simulink model "Noordergraaf_Rideout_2021b"  (R2021b)
settings: Solver=FixedStepAuto  StartTime=0.0  StopTime=stop_time  FixedStep=sample_time  RelTol=1e-3
undefined symbols (not defined in the file or in its folder): C, L, R, R_105, R_26, R_29, R_34, R_35, R_60, R_61, R_64, R_65, R_66, R_70, R_82, R_84, R_88, R_90, R_AT, R_SA, sample_time
libraries: ee_lib x421, fl_lib x87, nesl_utility x57, simulink x1
(part 1 of 9)
settings Model: Creator=jorge  LastModifiedBy=jorge
settings SolverCC: InitialStep=sample_time

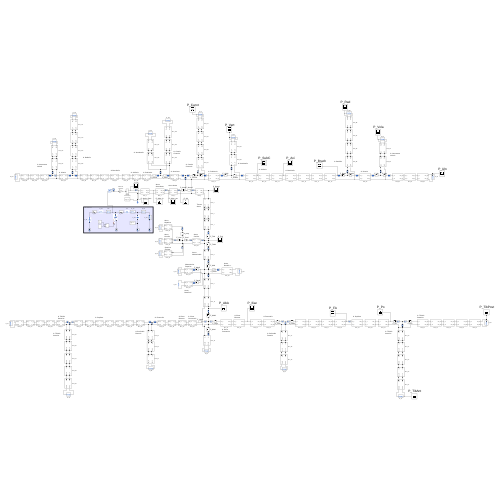
[thumbnail: Simulink's stored preview of the top-level diagram]
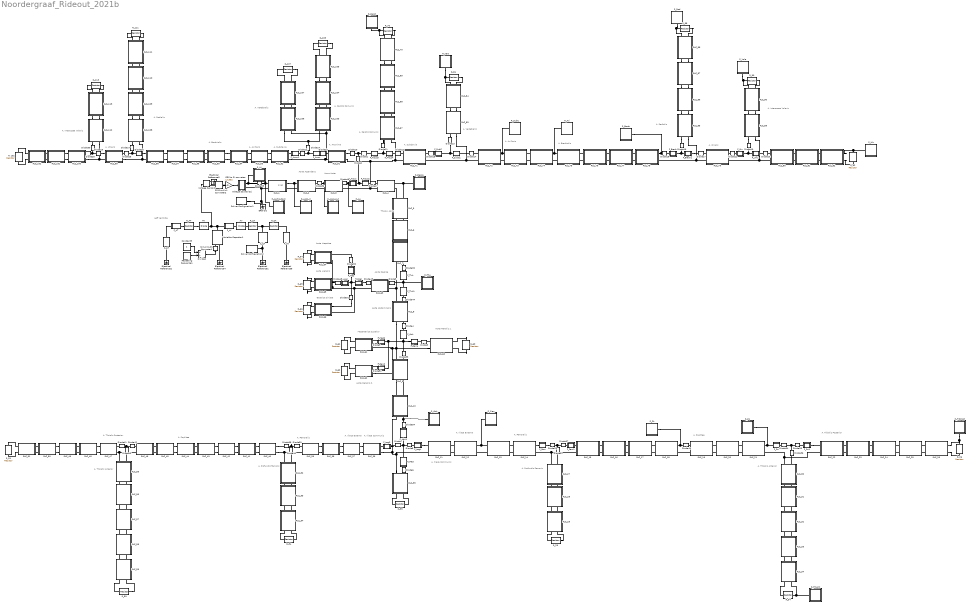
== system Noordergraaf_Rideout_2021b ==
  note: Aorta
      | Ascendens
  note: ones
  note: Arcus Aorta
  note: Thorax
      | Aorta
  note: Aorta
      | Coelica
  note: Gastrica
      | Sinistra
  note: Aorta
      | Lienalis
  note: Aorta
      | Hepatica
  note: Aorta
      | Abdominalis
  note: Aorta
      | Renalis d.
  note: Mesenterica
      | Superior
  note: Aorta
      | Renalis s.
  note: A. Iliaca
      | Communis
  note: A. Iliaca
      | Externa
  note: A. Femoralis
  note: A. Profundis
      | Femoris
  note: A. Tibialis
      | Anterior
  note: A. Poplitea
  note: A. Tibialis
      | Posterior
  note: A. Iliaca
      | Communis
  note: A. Iliaca
      | Externa
  note: A. Femoralis
  note: A. Poplitea
  note: A. Tibialis
      | Posterior
  note: A. Profundis
      | Femoris
  note: A. Tibialis
      | Anterior
  note: A. Carotis
      | Comunis
  note: A. Ulnaris
  note: A. Brachialis
  note: A. Subclavia
  note: A. Axillaris
  note: A. Radialis
  note: A. Subclavia
  note: A. Axillaris
  note: A. Brachialis
  note: A. Ulnaris
  note: A. Vertebralis
  note: A. Carotis
      | Comunis
  note: A. Vertebralis
  note: A. Interossea
      | Volaris
  note: A. Interossea
      | Volaris
  note: A. Radialis
  note: A. Anonima
  note: Left Ventricle
  " P_AA" : Subsystem
      settings: PortSchema="{\"entries\":[{\"content\":{\"sides\":[{\"content\":{\"connectorIds\":[]},\"type\":\"ConnectorPlacement.EquallySpacedRectSide\",\"uuid\":\"a76c572b-3baf-4a16-ab2f-87d419d93200\"},{\"content\":{\"connectorIds\":[],\"side\":\"RIGHT\"},\"type\":\"ConnectorPlacement.EquallySpacedRectSide\",\"uuid\":\"88de64cb-36a9-4b54-8774-bd24fb5aa84a\"},{\"content\":{\"connectorIds\":[\"LConn1\"],\"side\":\"TOP\"},\"type\":\"ConnectorPlacement.EquallySpacedRectSide\",\"uuid\":\"3a1c039d-3fc9-4c0f-9a54-0653a75cef5f\"},{\"content\":{\"connectorIds\":[],\"side\":\"HIDDEN\"},\"type\":\"ConnectorPlacement.EquallySpacedRectSide\",\"uuid\":\"5afc8217-ede4-4d55-8a13-208761f7f032\"}]},\"type\":\"ConnectorPlacement.EquallySpacedConnector\",\"uuid\":\"92a25d9f-67d7-41a2-ac65-068fc761adb7\"}],\"packageUris\":[\"http://schema.mathworks.com/mf0/Connector/R2020b\"],\"version\":\"1.0\"}"
      mask Display: image('$imagefile');
  " P_AAsc_in" : Subsystem
      settings: PortSchema="{\"entries\":[{\"content\":{\"sides\":[{\"content\":{\"connectorIds\":[]},\"type\":\"ConnectorPlacement.EquallySpacedRectSide\",\"uuid\":\"a76c572b-3baf-4a16-ab2f-87d419d93200\"},{\"content\":{\"connectorIds\":[],\"side\":\"RIGHT\"},\"type\":\"ConnectorPlacement.EquallySpacedRectSide\",\"uuid\":\"88de64cb-36a9-4b54-8774-bd24fb5aa84a\"},{\"content\":{\"connectorIds\":[\"LConn1\"],\"side\":\"TOP\"},\"type\":\"ConnectorPlacement.EquallySpacedRectSide\",\"uuid\":\"3a1c039d-3fc9-4c0f-9a54-0653a75cef5f\"},{\"content\":{\"connectorIds\":[],\"side\":\"HIDDEN\"},\"type\":\"ConnectorPlacement.EquallySpacedRectSide\",\"uuid\":\"5afc8217-ede4-4d55-8a13-208761f7f032\"}]},\"type\":\"ConnectorPlacement.EquallySpacedConnector\",\"uuid\":\"92a25d9f-67d7-41a2-ac65-068fc761adb7\"}],\"packageUris\":[\"http://schema.mathworks.com/mf0/Connector/R2020b\"],\"version\":\"1.0\"}"
      mask Display: image('$imagefile'); % Use "Edit Image" on toolstrip to change.
  " P_AAsc_out" : Subsystem
      settings: PortSchema="{\"entries\":[{\"content\":{\"sides\":[{\"content\":{\"connectorIds\":[]},\"type\":\"ConnectorPlacement.EquallySpacedRectSide\",\"uuid\":\"a76c572b-3baf-4a16-ab2f-87d419d93200\"},{\"content\":{\"connectorIds\":[],\"side\":\"RIGHT\"},\"type\":\"ConnectorPlacement.EquallySpacedRectSide\",\"uuid\":\"88de64cb-36a9-4b54-8774-bd24fb5aa84a\"},{\"content\":{\"connectorIds\":[\"LConn1\"],\"side\":\"TOP\"},\"type\":\"ConnectorPlacement.EquallySpacedRectSide\",\"uuid\":\"3a1c039d-3fc9-4c0f-9a54-0653a75cef5f\"},{\"content\":{\"connectorIds\":[],\"side\":\"HIDDEN\"},\"type\":\"ConnectorPlacement.EquallySpacedRectSide\",\"uuid\":\"5afc8217-ede4-4d55-8a13-208761f7f032\"}]},\"type\":\"ConnectorPlacement.EquallySpacedConnector\",\"uuid\":\"92a25d9f-67d7-41a2-ac65-068fc761adb7\"}],\"packageUris\":[\"http://schema.mathworks.com/mf0/Connector/R2020b\"],\"version\":\"1.0\"}"
      mask Display: image('$imagefile'); % Use "Edit Image" on toolstrip to change.
  " P_AbA" : Subsystem
      settings: PortSchema="{\"entries\":[{\"content\":{\"sides\":[{\"content\":{\"connectorIds\":[]},\"type\":\"ConnectorPlacement.EquallySpacedRectSide\",\"uuid\":\"a76c572b-3baf-4a16-ab2f-87d419d93200\"},{\"content\":{\"connectorIds\":[],\"side\":\"RIGHT\"},\"type\":\"ConnectorPlacement.EquallySpacedRectSide\",\"uuid\":\"88de64cb-36a9-4b54-8774-bd24fb5aa84a\"},{\"content\":{\"connectorIds\":[\"LConn1\"],\"side\":\"TOP\"},\"type\":\"ConnectorPlacement.EquallySpacedRectSide\",\"uuid\":\"3a1c039d-3fc9-4c0f-9a54-0653a75cef5f\"},{\"content\":{\"connectorIds\":[],\"side\":\"HIDDEN\"},\"type\":\"ConnectorPlacement.EquallySpacedRectSide\",\"uuid\":\"5afc8217-ede4-4d55-8a13-208761f7f032\"}]},\"type\":\"ConnectorPlacement.EquallySpacedConnector\",\"uuid\":\"92a25d9f-67d7-41a2-ac65-068fc761adb7\"}],\"packageUris\":[\"http://schema.mathworks.com/mf0/Connector/R2020b\"],\"version\":\"1.0\"}"
      mask Display: image('$imagefile'); % Use "Edit Image" on toolstrip to change.
  " P_Aortic_Root" : Subsystem
      settings: PortSchema="{\"entries\":[{\"content\":{\"sides\":[{\"content\":{\"connectorIds\":[]},\"type\":\"ConnectorPlacement.EquallySpacedRectSide\",\"uuid\":\"a76c572b-3baf-4a16-ab2f-87d419d93200\"},{\"content\":{\"connectorIds\":[],\"side\":\"RIGHT\"},\"type\":\"ConnectorPlacement.EquallySpacedRectSide\",\"uuid\":\"88de64cb-36a9-4b54-8774-bd24fb5aa84a\"},{\"content\":{\"connectorIds\":[\"LConn1\"],\"side\":\"TOP\"},\"type\":\"ConnectorPlacement.EquallySpacedRectSide\",\"uuid\":\"3a1c039d-3fc9-4c0f-9a54-0653a75cef5f\"},{\"content\":{\"connectorIds\":[],\"side\":\"HIDDEN\"},\"type\":\"ConnectorPlacement.EquallySpacedRectSide\",\"uuid\":\"5afc8217-ede4-4d55-8a13-208761f7f032\"}]},\"type\":\"ConnectorPlacement.EquallySpacedConnector\",\"uuid\":\"92a25d9f-67d7-41a2-ac65-068fc761adb7\"}],\"packageUris\":[\"http://schema.mathworks.com/mf0/Connector/R2020b\"],\"version\":\"1.0\"}"
      mask Display: image('$imagefile'); % Use "Edit Image" on toolstrip to change.
  " P_Axi" : Subsystem
      settings: PortSchema="{\"entries\":[{\"content\":{\"sides\":[{\"content\":{\"connectorIds\":[]},\"type\":\"ConnectorPlacement.EquallySpacedRectSide\",\"uuid\":\"a76c572b-3baf-4a16-ab2f-87d419d93200\"},{\"content\":{\"connectorIds\":[],\"side\":\"RIGHT\"},\"type\":\"ConnectorPlacement.EquallySpacedRectSide\",\"uuid\":\"88de64cb-36a9-4b54-8774-bd24fb5aa84a\"},{\"content\":{\"connectorIds\":[\"LConn1\"],\"side\":\"TOP\"},\"type\":\"ConnectorPlacement.EquallySpacedRectSide\",\"uuid\":\"3a1c039d-3fc9-4c0f-9a54-0653a75cef5f\"},{\"content\":{\"connectorIds\":[],\"side\":\"BOTTOM\"},\"type\":\"ConnectorPlacement.EquallySpacedRectSide\",\"uuid\":\"16f5eb9b-ee63-4f34-9118-7825bbfe571f\"},{\"content\":{\"connectorIds\":[],\"side\":\"HIDDEN\"},\"type\":\"ConnectorPlacement.EquallySpacedRectSide\",\"uuid\":\"5afc8217-ede4-4d55-8a13-208761f7f032\"}]},\"type\":\"ConnectorPlacement.EquallySpacedConnector\",\"uuid\":\"92a25d9f-67d7-41a2-ac65-068fc761adb7\"}],\"packageUris\":[\"http://schema.mathworks.com/mf0/Connector/R2020b\"],\"version\":\"1.0\"}"
      mask Display: image('$imagefile'); % Use "Edit Image" on toolstrip to change.
  " P_Brach" : Subsystem
      settings: PortSchema="{\"entries\":[{\"content\":{\"sides\":[{\"content\":{\"connectorIds\":[]},\"type\":\"ConnectorPlacement.EquallySpacedRectSide\",\"uuid\":\"a76c572b-3baf-4a16-ab2f-87d419d93200\"},{\"content\":{\"connectorIds\":[],\"side\":\"RIGHT\"},\"type\":\"ConnectorPlacement.EquallySpacedRectSide\",\"uuid\":\"88de64cb-36a9-4b54-8774-bd24fb5aa84a\"},{\"content\":{\"connectorIds\":[],\"side\":\"TOP\"},\"type\":\"ConnectorPlacement.EquallySpacedRectSide\",\"uuid\":\"3a1c039d-3fc9-4c0f-9a54-0653a75cef5f\"},{\"content\":{\"connectorIds\":[\"RConn1\"],\"side\":\"BOTTOM\"},\"type\":\"ConnectorPlacement.EquallySpacedRectSide\",\"uuid\":\"16f5eb9b-ee63-4f34-9118-7825bbfe571f\"},{\"content\":{\"connectorIds\":[],\"side\":\"HIDDEN\"},\"type\":\"ConnectorPlacement.EquallySpacedRectSide\",\"uuid\":\"5afc8217-ede4-4d55-8a13-208761f7f032\"}]},\"type\":\"ConnectorPlacement.EquallySpacedConnector\",\"uuid\":\"92a25d9f-67d7-41a2-ac65-068fc761adb7\"}],\"packageUris\":[\"http://schema.mathworks.com/mf0/Connector/R2020b\"],\"version\":\"1.0\"}"
      mask Display: image('$imagefile'); % Use "Edit Image" on toolstrip to change.
  " P_Carot" : Subsystem
      mask Display: image('$imagefile'); % Use "Edit Image" on toolstrip to change.
  " P_DescA" : Subsystem
      settings: PortSchema="{\"entries\":[{\"content\":{\"sides\":[{\"content\":{\"connectorIds\":[]},\"type\":\"ConnectorPlacement.EquallySpacedRectSide\",\"uuid\":\"a76c572b-3baf-4a16-ab2f-87d419d93200\"},{\"content\":{\"connectorIds\":[],\"side\":\"RIGHT\"},\"type\":\"ConnectorPlacement.EquallySpacedRectSide\",\"uuid\":\"88de64cb-36a9-4b54-8774-bd24fb5aa84a\"},{\"content\":{\"connectorIds\":[\"LConn1\"],\"side\":\"TOP\"},\"type\":\"ConnectorPlacement.EquallySpacedRectSide\",\"uuid\":\"3a1c039d-3fc9-4c0f-9a54-0653a75cef5f\"},{\"content\":{\"connectorIds\":[],\"side\":\"HIDDEN\"},\"type\":\"ConnectorPlacement.EquallySpacedRectSide\",\"uuid\":\"5afc8217-ede4-4d55-8a13-208761f7f032\"}]},\"type\":\"ConnectorPlacement.EquallySpacedConnector\",\"uuid\":\"92a25d9f-67d7-41a2-ac65-068fc761adb7\"}],\"packageUris\":[\"http://schema.mathworks.com/mf0/Connector/R2020b\"],\"version\":\"1.0\"}"
      mask Display: image('$imagefile'); % Use "Edit Image" on toolstrip to change.
  " P_FA" : Subsystem
      settings: PortSchema="{\"entries\":[{\"content\":{\"sides\":[{\"content\":{\"connectorIds\":[]},\"type\":\"ConnectorPlacement.EquallySpacedRectSide\",\"uuid\":\"a76c572b-3baf-4a16-ab2f-87d419d93200\"},{\"content\":{\"connectorIds\":[],\"side\":\"RIGHT\"},\"type\":\"ConnectorPlacement.EquallySpacedRectSide\",\"uuid\":\"88de64cb-36a9-4b54-8774-bd24fb5aa84a\"},{\"content\":{\"connectorIds\":[],\"side\":\"TOP\"},\"type\":\"ConnectorPlacement.EquallySpacedRectSide\",\"uuid\":\"3a1c039d-3fc9-4c0f-9a54-0653a75cef5f\"},{\"content\":{\"connectorIds\":[\"RConn1\"],\"side\":\"BOTTOM\"},\"type\":\"ConnectorPlacement.EquallySpacedRectSide\",\"uuid\":\"041fbf42-3c46-4830-b301-418dfd34a912\"},{\"content\":{\"connectorIds\":[],\"side\":\"HIDDEN\"},\"type\":\"ConnectorPlacement.EquallySpacedRectSide\",\"uuid\":\"5afc8217-ede4-4d55-8a13-208761f7f032\"}]},\"type\":\"ConnectorPlacement.EquallySpacedConnector\",\"uuid\":\"92a25d9f-67d7-41a2-ac65-068fc761adb7\"}],\"packageUris\":[\"http://schema.mathworks.com/mf0/Connector/R2020b\"],\"version\":\"1.0\"}"
      mask Display: image('$imagefile'); % Use "Edit Image" on toolstrip to change.
  " P_Iliac" : Subsystem
      settings: PortSchema="{\"entries\":[{\"content\":{\"sides\":[{\"content\":{\"connectorIds\":[]},\"type\":\"ConnectorPlacement.EquallySpacedRectSide\",\"uuid\":\"a76c572b-3baf-4a16-ab2f-87d419d93200\"},{\"content\":{\"connectorIds\":[],\"side\":\"RIGHT\"},\"type\":\"ConnectorPlacement.EquallySpacedRectSide\",\"uuid\":\"88de64cb-36a9-4b54-8774-bd24fb5aa84a\"},{\"content\":{\"connectorIds\":[\"LConn1\"],\"side\":\"TOP\"},\"type\":\"ConnectorPlacement.EquallySpacedRectSide\",\"uuid\":\"3a1c039d-3fc9-4c0f-9a54-0653a75cef5f\"},{\"content\":{\"connectorIds\":[],\"side\":\"BOTTOM\"},\"type\":\"ConnectorPlacement.EquallySpacedRectSide\",\"uuid\":\"041fbf42-3c46-4830-b301-418dfd34a912\"},{\"content\":{\"connectorIds\":[],\"side\":\"HIDDEN\"},\"type\":\"ConnectorPlacement.EquallySpacedRectSide\",\"uuid\":\"5afc8217-ede4-4d55-8a13-208761f7f032\"}]},\"type\":\"ConnectorPlacement.EquallySpacedConnector\",\"uuid\":\"92a25d9f-67d7-41a2-ac65-068fc761adb7\"}],\"packageUris\":[\"http://schema.mathworks.com/mf0/Connector/R2020b\"],\"version\":\"1.0\"}"
      mask Display: image('$imagefile'); % Use "Edit Image" on toolstrip to change.
  " P_LV" : Subsystem
      settings: PortSchema="{\"entries\":[{\"content\":{\"sides\":[{\"content\":{\"connectorIds\":[]},\"type\":\"ConnectorPlacement.EquallySpacedRectSide\",\"uuid\":\"a76c572b-3baf-4a16-ab2f-87d419d93200\"},{\"content\":{\"connectorIds\":[],\"side\":\"RIGHT\"},\"type\":\"ConnectorPlacement.EquallySpacedRectSide\",\"uuid\":\"88de64cb-36a9-4b54-8774-bd24fb5aa84a\"},{\"content\":{\"connectorIds\":[\"LConn1\"],\"side\":\"TOP\"},\"type\":\"ConnectorPlacement.EquallySpacedRectSide\",\"uuid\":\"3a1c039d-3fc9-4c0f-9a54-0653a75cef5f\"},{\"content\":{\"connectorIds\":[],\"side\":\"HIDDEN\"},\"type\":\"ConnectorPlacement.EquallySpacedRectSide\",\"uuid\":\"5afc8217-ede4-4d55-8a13-208761f7f032\"}]},\"type\":\"ConnectorPlacement.EquallySpacedConnector\",\"uuid\":\"92a25d9f-67d7-41a2-ac65-068fc761adb7\"}],\"packageUris\":[\"http://schema.mathworks.com/mf0/Connector/R2020b\"],\"version\":\"1.0\"}"
      mask Display: image('$imagefile'); % Use "Edit Image" on toolstrip to change.
  " P_Po" : Subsystem
      settings: PortSchema="{\"entries\":[{\"content\":{\"sides\":[{\"content\":{\"connectorIds\":[]},\"type\":\"ConnectorPlacement.EquallySpacedRectSide\",\"uuid\":\"a76c572b-3baf-4a16-ab2f-87d419d93200\"},{\"content\":{\"connectorIds\":[],\"side\":\"RIGHT\"},\"type\":\"ConnectorPlacement.EquallySpacedRectSide\",\"uuid\":\"88de64cb-36a9-4b54-8774-bd24fb5aa84a\"},{\"content\":{\"connectorIds\":[],\"side\":\"TOP\"},\"type\":\"ConnectorPlacement.EquallySpacedRectSide\",\"uuid\":\"3a1c039d-3fc9-4c0f-9a54-0653a75cef5f\"},{\"content\":{\"connectorIds\":[\"RConn1\"],\"side\":\"BOTTOM\"},\"type\":\"ConnectorPlacement.EquallySpacedRectSide\",\"uuid\":\"041fbf42-3c46-4830-b301-418dfd34a912\"},{\"content\":{\"connectorIds\":[],\"side\":\"HIDDEN\"},\"type\":\"ConnectorPlacement.EquallySpacedRectSide\",\"uuid\":\"5afc8217-ede4-4d55-8a13-208761f7f032\"}]},\"type\":\"ConnectorPlacement.EquallySpacedConnector\",\"uuid\":\"92a25d9f-67d7-41a2-ac65-068fc761adb7\"}],\"packageUris\":[\"http://schema.mathworks.com/mf0/Connector/R2020b\"],\"version\":\"1.0\"}"
      mask Display: image('$imagefile'); % Use "Edit Image" on toolstrip to change.
  " P_Rad" : Subsystem
      mask Display: image('$imagefile'); % Use "Edit Image" on toolstrip to change.
  " P_SubC" : Subsystem
      settings: PortSchema="{\"entries\":[{\"content\":{\"sides\":[{\"content\":{\"connectorIds\":[]},\"type\":\"ConnectorPlacement.EquallySpacedRectSide\",\"uuid\":\"a76c572b-3baf-4a16-ab2f-87d419d93200\"},{\"content\":{\"connectorIds\":[],\"side\":\"RIGHT\"},\"type\":\"ConnectorPlacement.EquallySpacedRectSide\",\"uuid\":\"88de64cb-36a9-4b54-8774-bd24fb5aa84a\"},{\"content\":{\"connectorIds\":[\"LConn1\"],\"side\":\"TOP\"},\"type\":\"ConnectorPlacement.EquallySpacedRectSide\",\"uuid\":\"3a1c039d-3fc9-4c0f-9a54-0653a75cef5f\"},{\"content\":{\"connectorIds\":[],\"side\":\"BOTTOM\"},\"type\":\"ConnectorPlacement.EquallySpacedRectSide\",\"uuid\":\"16f5eb9b-ee63-4f34-9118-7825bbfe571f\"},{\"content\":{\"connectorIds\":[],\"side\":\"HIDDEN\"},\"type\":\"ConnectorPlacement.EquallySpacedRectSide\",\"uuid\":\"5afc8217-ede4-4d55-8a13-208761f7f032\"}]},\"type\":\"ConnectorPlacement.EquallySpacedConnector\",\"uuid\":\"92a25d9f-67d7-41a2-ac65-068fc761adb7\"}],\"packageUris\":[\"http://schema.mathworks.com/mf0/Connector/R2020b\"],\"version\":\"1.0\"}"
      mask Display: image('$imagefile'); % Use "Edit Image" on toolstrip to change.
  " P_ThA" : Subsystem
      settings: PortSchema="{\"entries\":[{\"content\":{\"sides\":[{\"content\":{\"connectorIds\":[]},\"type\":\"ConnectorPlacement.EquallySpacedRectSide\",\"uuid\":\"a76c572b-3baf-4a16-ab2f-87d419d93200\"},{\"content\":{\"connectorIds\":[],\"side\":\"RIGHT\"},\"type\":\"ConnectorPlacement.EquallySpacedRectSide\",\"uuid\":\"88de64cb-36a9-4b54-8774-bd24fb5aa84a\"},{\"content\":{\"connectorIds\":[\"LConn1\"],\"side\":\"TOP\"},\"type\":\"ConnectorPlacement.EquallySpacedRectSide\",\"uuid\":\"3a1c039d-3fc9-4c0f-9a54-0653a75cef5f\"},{\"content\":{\"connectorIds\":[],\"side\":\"HIDDEN\"},\"type\":\"ConnectorPlacement.EquallySpacedRectSide\",\"uuid\":\"5afc8217-ede4-4d55-8a13-208761f7f032\"}]},\"type\":\"ConnectorPlacement.EquallySpacedConnector\",\"uuid\":\"92a25d9f-67d7-41a2-ac65-068fc761adb7\"}],\"packageUris\":[\"http://schema.mathworks.com/mf0/Connector/R2020b\"],\"version\":\"1.0\"}"
      mask Display: image('$imagefile'); % Use "Edit Image" on toolstrip to change.
  " P_TibAnt" : Subsystem
      settings: PortSchema="{\"entries\":[{\"content\":{\"sides\":[{\"content\":{\"connectorIds\":[]},\"type\":\"ConnectorPlacement.EquallySpacedRectSide\",\"uuid\":\"efa007d6-45f4-4edc-b08d-571edfadacea\"},{\"content\":{\"connectorIds\":[],\"side\":\"RIGHT\"},\"type\":\"ConnectorPlacement.EquallySpacedRectSide\",\"uuid\":\"9590d5ff-e9bb-4f62-8234-4beabe73ec5b\"},{\"content\":{\"connectorIds\":[\"LConn1\"],\"side\":\"TOP\"},\"type\":\"ConnectorPlacement.EquallySpacedRectSide\",\"uuid\":\"6b36768b-9c7e-47c9-8a74-9f42572fa7f1\"}]},\"type\":\"ConnectorPlacement.EquallySpacedConnector\",\"uuid\":\"e0d20f9b-b643-4fc3-baf2-1c11480af55a\"}],\"packageUris\":[\"http://schema.mathworks.com/mf0/Connector/R2020b\"],\"version\":\"1.0\"}"
      mask Display: image('$imagefile'); % Use "Edit Image" on toolstrip to change.
  " P_TibPost" : Subsystem
      mask Display: image('$imagefile'); % Use "Edit Image" on toolstrip to change.
  " P_Uln" : Subsystem
      settings: PortSchema="{\"entries\":[{\"content\":{\"sides\":[{\"content\":{\"connectorIds\":[]},\"type\":\"ConnectorPlacement.EquallySpacedRectSide\",\"uuid\":\"a76c572b-3baf-4a16-ab2f-87d419d93200\"},{\"content\":{\"connectorIds\":[],\"side\":\"RIGHT\"},\"type\":\"ConnectorPlacement.EquallySpacedRectSide\",\"uuid\":\"88de64cb-36a9-4b54-8774-bd24fb5aa84a\"},{\"content\":{\"connectorIds\":[\"LConn1\"],\"side\":\"TOP\"},\"type\":\"ConnectorPlacement.EquallySpacedRectSide\",\"uuid\":\"3a1c039d-3fc9-4c0f-9a54-0653a75cef5f\"},{\"content\":{\"connectorIds\":[],\"side\":\"BOTTOM\"},\"type\":\"ConnectorPlacement.EquallySpacedRectSide\",\"uuid\":\"16f5eb9b-ee63-4f34-9118-7825bbfe571f\"},{\"content\":{\"connectorIds\":[],\"side\":\"HIDDEN\"},\"type\":\"ConnectorPlacement.EquallySpacedRectSide\",\"uuid\":\"5afc8217-ede4-4d55-8a13-208761f7f032\"}]},\"type\":\"ConnectorPlacement.EquallySpacedConnector\",\"uuid\":\"92a25d9f-67d7-41a2-ac65-068fc761adb7\"}],\"packageUris\":[\"http://schema.mathworks.com/mf0/Connector/R2020b\"],\"version\":\"1.0\"}"
      mask Display: image('$imagefile'); % Use "Edit Image" on toolstrip to change.
  " P_Vert" : Subsystem
      mask Display: image('$imagefile'); % Use "Edit Image" on toolstrip to change.
  " P_Vola" : Subsystem
      mask Display: image('$imagefile'); % Use "Edit Image" on toolstrip to change.
  AV : fl_lib/Electrical/Electrical Elements/Diode  Vf=1 V  Ron=10^(-3) Ohm  Goff=1e-8 1/Ohm  i_specify=off  i_priority=None  i=0 A  i_nominal_specify=off  i_nominal_unit=A  i_nominal_value=1  v_specify=off  v_priority=None  v=0 V  v_nominal_specify=off  v_nominal_unit=V  v_nominal_value=1
  CGS to SI converter : Gain  Gain=1/1332
  C_CA : fl_lib/Electrical/Electrical Elements/Capacitor  c=C_CA F  r=0 Ohm  g=0 1/Ohm  i_specify=off  i_priority=None  i=0 A  i_nominal_specify=off  i_nominal_unit=A  i_nominal_value=220  v_specify=off  v_priority=None  v=0 V  v_nominal_specify=off  v_nominal_unit=V  v_nominal_value=1  vc_specify=off  vc_priority=High  vc=0 V  vc_nominal_specify=off  vc_nominal_unit=V  vc_nominal_value=1
  Constant5 : Constant  SampleTime=sample_time
  Diode{1..56} (56 alike) : ee_lib/Semiconductors & Converters/Diode  ModelType=ee.enum.diode.modelType.pwl  TableType=ee.enum.diode.tableType.IfMat  IfMat=[.07, .12, .19, 1.75, 4.24, 7.32, 11.2; .16, .3, .72, 2.14, 5.02, 8.35, 13.12] A  VfMat=[.9, 1.15, 1.25, 1.5, 1.75, 2.17, 2.6, 2.85; .58, .68, .75, 1.1, 1.38, 1.77, 2.27, 2.7] V  TjVec=[25, 125] degC  VfVec=[.5, .7, .9, 1.3, 1.7, 2.1, 2.5] V  IfVec=[.1, .2, .5, 1, 2, 4, 7, 10] A  Vf=0.6 V  Ron=0.3 Ohm  Goff=1e-8 S  prmExp=ee.enum.diode.expParam.useTwo  I12=[.0137, .545] A  V12=[.6, .7] V  RS=0 Ohm  Tmeas=25 degC  IS=1e-12 A  ec=1  I1=0.0137 A  V1=0.6 V  N_series=1  N_parallel=1  ZenerEnable=false  Rz=0.3 Ohm  BV=inf V  C_param=ee.enum.diode.capParam.fixed  CJ=5 pF  CJ0=5 pF  Vvec=[.1, 10, 100] V  Cvec=[3.5, 1, .4] pF  VJ=1 V  Mgrad=0.5  FC=0.5  Q_param=ee.enum.diode.recoveryParam.off  iRM=-7.15 A  iF=4 A  didt=-750 A/us  trr_factor=3  trr=115 ns  Qrr=150 nA*s  Vr=-600 V  Ls=150 nH  Erec=0.03 J  TT=50 ns  tau=100 ns  T_param=ee.enum.diode.temperatureParam.off  Tdevice=25 degC  I1_T2=0.245 A  V1_T2=0.5 V  IS_T2=1.25e-7 A  Tmeas2=125 degC  XTI_param=ee.enum.diode.xtiParam.pn  XTI=3  EG_param=ee.enum.diode.egapParam.material_si  EG=1.11 eV  dBVdT=0 V/K  enable_faults=ee.enum.enable.no  fault_action=simscape.enum.assert.action.none  fault_types=ee.enum.diode.faults.open  tau_fault=1e-3 s  IfMat_faulted=[.07, .12, .19, 1.75, 4.24, 7.32, 11.2; .16, .3, .72, 2.14, 4.02, 6.35, 9.12] A  VfMat_faulted=[.9, 1.15, 1.25, 1.5, 1.75, 2.17, 2.6, 2.85; .58, .68, .75, 1.1, 1.38, 1.77, 2.27, 2.7] V  VfVec_faulted=[.5, .7, .9, 1.3, 1.7, 2.1, 2.5] V  IfVec_faulted=[.1, .2, .5, 1, 2, 4, 7, 10] A  Ropen_faulted=1000 Ohm  Gshort_faulted=1000 1/Ohm  Vf_faulted=0.6 V  Ron_faulted=0.3 Ohm  Goff_faulted=1e-8 S  I12_faulted=[.0137, .545] A  V12_faulted=[.6, .7] V  IS_faulted=1e-12 A  ec_faulted=1  I1_faulted=0.0137 A  V1_faulted=0.6 V  RS_faulted=0 Ohm  Rz_faulted=0.3 Ohm  BV_faulted=inf V  Cscale_faulted=100  fault_trigger=ee.enum.faults.faultTrigger.temporal  t_fault=inf s  max_permissible_voltage=inf V  n_fail_on_voltage=1  max_permissible_current=inf A  t_fail_on_current=1 s  max_permissible_dVdt=inf V/s  enable_fault_input=simscape.enum.onoff.off  i_specify=off  i_priority=None  i=0 A  i_nominal_specify=off  i_nominal_unit=A  i_nominal_value=1  v_specify=off  v_priority=None  v=0 V  v_nominal_specify=off  v_nominal_unit=V  v_nominal_value=1  v_capacitor_specify=off  v_capacitor_priority=None  v_capacitor=0 V  v_capacitor_nominal_specify=off  v_capacitor_nominal_unit=V  v_capacitor_nominal_value=1  faulted_specify=off  faulted_priority=None  faulted=0  faulted_nominal_specify=off  faulted_nominal_unit=1  faulted_nominal_value=1  i_diode_specify=off  i_diode_priority=None  i_diode=0 A  i_diode_nominal_specify=off  i_diode_nominal_unit=A  i_diode_nominal_value=1  v_diode_specify=off  v_diode_priority=None  v_diode=0 V  v_diode_nominal_specify=off  v_diode_nominal_unit=V  v_diode_nominal_value=1  i_capacitor_specify=off  i_capacitor_priority=None  i_capacitor=0 A  i_capacitor_nominal_specify=off  i_capacitor_nominal_unit=A  i_capacitor_nominal_value=1  power_dissipated_specify=off  power_dissipated_priority=None  power_dissipated=0 W  power_dissipated_nominal_specify=off  power_dissipated_nominal_unit=W  power_dissipated_nominal_value=1  fidelity_level=ee.enum.diode.fidelity.includeChargeDyn  rec_loss_model=ee.enum.diode.reverseRecoveryModel.fixed  ErecVal=0 J  scaleWithIandV=true  ErecMat=zeros(2, 3) J  TjrecVec=[298.15, 398.15] K  IfrecVec=[.1, 1, 10] A  IrecVal=10 A  VrecVal=10 V  tFilter=1 / 1000 / 100 s  max_permissible_temperature=inf K  t_fail_on_temperature=1 s  thermal_network_parameterization=ee.enum.thermalNetworkTopology.junctionCase  Rth=[0, 10] K/W  Rth_Cauer=[1, 3, 10] K/W  Rth_Foster=[4, 6] K/W  thermal_mass_parameterization=ee.enum.thermalNetwork.timeconstant  thermal_mass=[0, 1] J/K  thermal_mass_Cauer=[.1, .3, 1] J/K  thermal_mass_Foster=[1.5, 3] J/K  thermal_time_constant=[0, 10] s  thermal_time_constant_Cauer=[1, 3, 10] s  thermal_time_constant_Foster=[6, 18] s  thermal_mass_initial_temperatures=[25, 25] degC  thermal_mass_initial_temperatures_Cauer=[25, 25, 25] degC  junction_thermal_mass=0.01 J/K  Tvec_initial_Foster=[25, 25, 25, 25] degC  no_thermal_network=0  junction_temperature_specify=off  junction_temperature_priority=None  junction_temperature=25 degC  junction_temperature_nominal_specify=off  junction_temperature_nominal_unit=degC  junction_temperature_nominal_value=1
  Divide2 : Product  Inputs=*/
  ERef Src : fl_lib/Electrical/Electrical Elements/Electrical Reference
  Electrical Reference{1..2,4..5,8} (5 alike) : fl_lib/Electrical/Electrical Elements/Electrical Reference
  F_AT : Subsystem
      mask Display: image('$imagefile'); % Use "Edit Image" on toolstrip to change.
  F_AbA : Subsystem
      mask Display: image('$imagefile'); % Use "Edit Image" on toolstrip to change.
  F_AbA1 : Subsystem
      mask Display: image('$imagefile'); % Use "Edit Image" on toolstrip to change.
  F_Anon : Subsystem
      mask Display: image('$imagefile'); % Use "Edit Image" on toolstrip to change.
  F_Anon1 : Subsystem
      mask Display: image('$imagefile'); % Use "Edit Image" on toolstrip to change.
  F_Arcus : Subsystem
      mask Display: image('$imagefile'); % Use "Edit Image" on toolstrip to change.
  F_Arcus2 : Subsystem
      mask Display: image('$imagefile'); % Use "Edit Image" on toolstrip to change.
  F_Arcus3 : Subsystem
      mask Display: image('$imagefile'); % Use "Edit Image" on toolstrip to change.
  F_Arcus4 : Subsystem
      mask Display: image('$imagefile'); % Use "Edit Image" on toolstrip to change.
  F_Brach : Subsystem
      mask Display: image('$imagefile'); % Use "Edit Image" on toolstrip to change.
  F_Brach1 : Subsystem
      mask Display: image('$imagefile'); % Use "Edit Image" on toolstrip to change.
  F_Coel : Subsystem
      mask Display: image('$imagefile'); % Use "Edit Image" on toolstrip to change.
  F_Fem : Subsystem
      mask Display: image('$imagefile'); % Use "Edit Image" on toolstrip to change.
  F_Fem1 : Subsystem
      mask Display: image('$imagefile'); % Use "Edit Image" on toolstrip to change.
  F_Hep : Subsystem
      mask Display: image('$imagefile'); % Use "Edit Image" on toolstrip to change.
  F_LV : Subsystem
      mask Display: image('$imagefile'); % Use "Edit Image" on toolstrip to change.
  F_LegL : Subsystem
      mask Display: image('$imagefile'); % Use "Edit Image" on toolstrip to change.
  F_LegR : Subsystem
      mask Display: image('$imagefile'); % Use "Edit Image" on toolstrip to change.
  F_Lien : Subsystem
      mask Display: image('$imagefile'); % Use "Edit Image" on toolstrip to change.
  F_MesI : Subsystem
      mask Display: image('$imagefile'); % Use "Edit Image" on toolstrip to change.
  F_MesS : Subsystem
      mask Display: image('$imagefile'); % Use "Edit Image" on toolstrip to change.
  F_Po : Subsystem
      mask Display: image('$imagefile'); % Use "Edit Image" on toolstrip to change.
  F_Po1 : Subsystem
      mask Display: image('$imagefile'); % Use "Edit Image" on toolstrip to change.
  F_Rena : Subsystem
      mask Display: image('C:\Users\jorge\Documents\papers\nanocom2021markov\matlab_code\icon_images\amper_H.png'); % Use "Edit Image" on toolstrip to change.
  F_Rend : Subsystem
      mask Display: image('$imagefile'); % Use "Edit Image" on toolstrip to change.
  F_SubC : Subsystem
      mask Display: image('$imagefile'); % Use "Edit Image" on toolstrip to change.
  F_SubC1 : Subsystem
      mask Display: image('$imagefile'); % Use "Edit Image" on toolstrip to change.
  F_ThA : Subsystem
      mask Display: image('$imagefile'); % Use "Edit Image" on toolstrip to change.
  F_ThA1 : Subsystem
      mask Display: image('$imagefile'); % Use "Edit Image" on toolstrip to change.
  F_Uln : Subsystem
      mask Display: image('$imagefile'); % Use "Edit Image" on toolstrip to change.
  F_Uln1 : Subsystem
      mask Display: image('$imagefile'); % Use "Edit Image" on toolstrip to change.
  MV : fl_lib/Electrical/Electrical Elements/Diode  Vf=1 V  Ron=10^(-3) Ohm  Goff=1e-8 1/Ohm  i_specify=off  i_priority=None  i=0 A  i_nominal_specify=off  i_nominal_unit=A  i_nominal_value=1  v_specify=off  v_priority=None  v=0 V  v_nominal_specify=off  v_nominal_unit=V  v_nominal_value=1
  PS-Simulink Converter2 : nesl_utility/PS-Simulink Converter  PhysicalDomain=network_engine_domain  SubClassName=ps_output  LeftPortType=input  RightPortType=output  PseudoPeriodic=off  Frequencies=[]  VectorFormat=1-D array  Unit=1  AffineConversion=off
  P_AT : ee_lib/Sources/Voltage Source  dc_voltage=P_AT V  ac_voltage=0 V  ac_shift=0 rad  ac_frequency=60 Hz  noise_mode=ee.enum.sources.noise.Disabled  PSD=0 V^2/Hz  sample_time=1e-3 s  repeatability=ee.enum.sources.repeatability.NotRepeatable  user_seed=0  auto_seed=2715962282  i_specify=off  i_priority=None  i=0 A  i_nominal_specify=off  i_nominal_unit=A  i_nominal_value=1  v_specify=off  v_priority=None  v=0 V  v_nominal_specify=off  v_nominal_unit=V  v_nominal_value=1
  P_SV : ee_lib/Sources/Voltage Source  dc_voltage=P_SV V  ac_voltage=0 V  ac_shift=0 rad  ac_frequency=60 Hz  noise_mode=ee.enum.sources.noise.Disabled  PSD=0 V^2/Hz  sample_time=1e-3 s  repeatability=ee.enum.sources.repeatability.NotRepeatable  user_seed=0  auto_seed=418932850  i_specify=off  i_priority=None  i=0 A  i_nominal_specify=off  i_nominal_unit=A  i_nominal_value=1  v_specify=off  v_priority=None  v=0 V  v_nominal_specify=off  v_nominal_unit=V  v_nominal_value=1
  RLC_1 : Subsystem  mask{R=R(1), L=L(1), C=C(1)}
  RLC_10 : Subsystem  mask{R=R(10), L=L(10), C=C(10)}
      settings: PortSchema="{\"entries\":[{\"content\":{\"sides\":[{\"content\":{\"connectorIds\":[]},\"type\":\"ConnectorPlacement.EquallySpacedRectSide\",\"uuid\":\"60dc27b1-37aa-45ee-bf60-4a562adeaebe\"},{\"content\":{\"connectorIds\":[],\"side\":\"RIGHT\"},\"type\":\"ConnectorPlacement.EquallySpacedRectSide\",\"uuid\":\"71f27a35-0868-434d-9527-40ce9dc69a44\"},{\"content\":{\"connectorIds\":[\"LConn1\",\"LConn2\"],\"side\":\"TOP\"},\"type\":\"ConnectorPlacement.EquallySpacedRectSide\",\"uuid\":\"3c3d5018-dce6-49a5-a481-da9d1bef79f3\"},{\"content\":{\"connectorIds\":[\"RConn1\",\"RConn2\"],\"side\":\"BOTTOM\"},\"type\":\"ConnectorPlacement.EquallySpacedRectSide\",\"uuid\":\"784ed6f0-011d-4b8b-967f-9fa51b650c0c\"}]},\"type\":\"ConnectorPlacement.EquallySpacedConnector\",\"uuid\":\"e53138d9-4137-42d6-a542-1330f1bd4428\"}],\"packageUris\":[\"http://schema.mathworks.com/mf0/Connector/R2020b\"],\"version\":\"1.0\"}"
  RLC_100 : Subsystem  mask{R=R(80), L=L(80), C=C(80)}
  RLC_101 : Subsystem  mask{R=R(81), L=L(81), C=C(81)}
  RLC_102 : Subsystem  mask{R=R(82), L=L(82), C=C(82)}
  RLC_103 : Subsystem  mask{R=R(103), L=L(103), C=C(103)}
  RLC_104 : Subsystem  mask{R=R(104), L=L(104), C=C(104)}
  RLC_105 : Subsystem  mask{R=R(105), L=L(105), C=C(105)}
  RLC_106 : Subsystem  mask{R=R(83), L=L(83), C=C(83)}
  RLC_107 : Subsystem  mask{R=R(84), L=L(84), C=C(84)}
  RLC_108 : Subsystem  mask{R=R(85), L=L(85), C=C(85)}
  RLC_109 : Subsystem  mask{R=R(86), L=L(86), C=C(86)}
  RLC_11 : Subsystem  mask{R=R(11), L=L(11), C=C(11)}
  RLC_110 : Subsystem  mask{R=R(87), L=L(87), C=C(87)}
  RLC_111 : Subsystem  mask{R=R(88), L=L(88), C=C(88)}
  RLC_112 : Subsystem  mask{R=R(89), L=L(89), C=C(89)}
  RLC_113 : Subsystem  mask{R=R(90), L=L(90), C=C(90)}
  RLC_12 : Subsystem  mask{R=R(12), L=L(12), C=C(12)}
  RLC_13 : Subsystem  mask{R=R(13), L=L(13), C=C(13)}
  RLC_14 : Subsystem  mask{R=R(14), L=L(14), C=C(14)}
  RLC_15 : Subsystem  mask{R=R(15), L=L(15), C=C(15)}
  RLC_16 : Subsystem  mask{R=R(16), L=L(16), C=C(16)}
  RLC_17 : Subsystem  mask{R=R(17), L=L(17), C=C(17)}
  RLC_18 : Subsystem  mask{R=R(18), L=L(18), C=C(18)}
  RLC_19 : Subsystem  mask{R=R(19), L=L(19), C=C(19)}
  RLC_2 : Subsystem  mask{R=R(2), L=L(2), C=C(2)}
  RLC_20 : Subsystem  mask{R=R(20), L=L(20), C=C(20)}
  RLC_21 : Subsystem  mask{R=R(21), L=L(21), C=C(21)}
  RLC_22 : Subsystem  mask{R=R(22), L=L(22), C=C(22)}
  RLC_23 : Subsystem  mask{R=R(23), L=L(23), C=C(23)}
  RLC_24 : Subsystem  mask{R=R(24), L=L(24), C=C(24)}
  RLC_25 : Subsystem  mask{R=R(25), L=L(25), C=C(25)}
  RLC_26 : Subsystem  mask{R=R(26), L=L(26), C=C(26)}
  RLC_27 : Subsystem  mask{R=R(27), L=L(27), C=C(27)}
      settings: PortSchema="{\"entries\":[{\"content\":{\"sides\":[{\"content\":{\"connectorIds\":[]},\"type\":\"ConnectorPlacement.EquallySpacedRectSide\",\"uuid\":\"60dc27b1-37aa-45ee-bf60-4a562adeaebe\"},{\"content\":{\"connectorIds\":[],\"side\":\"RIGHT\"},\"type\":\"ConnectorPlacement.EquallySpacedRectSide\",\"uuid\":\"71f27a35-0868-434d-9527-40ce9dc69a44\"},{\"content\":{\"connectorIds\":[\"LConn1\",\"LConn2\"],\"side\":\"TOP\"},\"type\":\"ConnectorPlacement.EquallySpacedRectSide\",\"uuid\":\"3c3d5018-dce6-49a5-a481-da9d1bef79f3\"},{\"content\":{\"connectorIds\":[\"RConn1\",\"RConn2\"],\"side\":\"BOTTOM\"},\"type\":\"ConnectorPlacement.EquallySpacedRectSide\",\"uuid\":\"784ed6f0-011d-4b8b-967f-9fa51b650c0c\"}]},\"type\":\"ConnectorPlacement.EquallySpacedConnector\",\"uuid\":\"e53138d9-4137-42d6-a542-1330f1bd4428\"}],\"packageUris\":[\"http://schema.mathworks.com/mf0/Connector/R2020b\"],\"version\":\"1.0\"}"
  RLC_28 : Subsystem  mask{R=R(28), L=L(28), C=C(28)}
      settings: PortSchema="{\"entries\":[{\"content\":{\"sides\":[{\"content\":{\"connectorIds\":[]},\"type\":\"ConnectorPlacement.EquallySpacedRectSide\",\"uuid\":\"60dc27b1-37aa-45ee-bf60-4a562adeaebe\"},{\"content\":{\"connectorIds\":[],\"side\":\"RIGHT\"},\"type\":\"ConnectorPlacement.EquallySpacedRectSide\",\"uuid\":\"71f27a35-0868-434d-9527-40ce9dc69a44\"},{\"content\":{\"connectorIds\":[\"LConn1\",\"LConn2\"],\"side\":\"TOP\"},\"type\":\"ConnectorPlacement.EquallySpacedRectSide\",\"uuid\":\"3c3d5018-dce6-49a5-a481-da9d1bef79f3\"},{\"content\":{\"connectorIds\":[\"RConn1\",\"RConn2\"],\"side\":\"BOTTOM\"},\"type\":\"ConnectorPlacement.EquallySpacedRectSide\",\"uuid\":\"784ed6f0-011d-4b8b-967f-9fa51b650c0c\"}]},\"type\":\"ConnectorPlacement.EquallySpacedConnector\",\"uuid\":\"e53138d9-4137-42d6-a542-1330f1bd4428\"}],\"packageUris\":[\"http://schema.mathworks.com/mf0/Connector/R2020b\"],\"version\":\"1.0\"}"
  RLC_29 : Subsystem  mask{R=R(29), L=L(29), C=C(29)}
      settings: PortSchema="{\"entries\":[{\"content\":{\"sides\":[{\"content\":{\"connectorIds\":[]},\"type\":\"ConnectorPlacement.EquallySpacedRectSide\",\"uuid\":\"60dc27b1-37aa-45ee-bf60-4a562adeaebe\"},{\"content\":{\"connectorIds\":[],\"side\":\"RIGHT\"},\"type\":\"ConnectorPlacement.EquallySpacedRectSide\",\"uuid\":\"71f27a35-0868-434d-9527-40ce9dc69a44\"},{\"content\":{\"connectorIds\":[\"LConn1\",\"LConn2\"],\"side\":\"TOP\"},\"type\":\"ConnectorPlacement.EquallySpacedRectSide\",\"uuid\":\"3c3d5018-dce6-49a5-a481-da9d1bef79f3\"},{\"content\":{\"connectorIds\":[\"RConn1\",\"RConn2\"],\"side\":\"BOTTOM\"},\"type\":\"ConnectorPlacement.EquallySpacedRectSide\",\"uuid\":\"784ed6f0-011d-4b8b-967f-9fa51b650c0c\"}]},\"type\":\"ConnectorPlacement.EquallySpacedConnector\",\"uuid\":\"e53138d9-4137-42d6-a542-1330f1bd4428\"}],\"packageUris\":[\"http://schema.mathworks.com/mf0/Connector/R2020b\"],\"version\":\"1.0\"}"
  RLC_3 : Subsystem  mask{R=R(3), L=L(3), C=C(3)}
  RLC_30 : Subsystem  mask{R=R(30), L=L(30), C=C(30)}
      settings: PortSchema="{\"entries\":[{\"content\":{\"sides\":[{\"content\":{\"connectorIds\":[]},\"type\":\"ConnectorPlacement.EquallySpacedRectSide\",\"uuid\":\"60dc27b1-37aa-45ee-bf60-4a562adeaebe\"},{\"content\":{\"connectorIds\":[],\"side\":\"RIGHT\"},\"type\":\"ConnectorPlacement.EquallySpacedRectSide\",\"uuid\":\"71f27a35-0868-434d-9527-40ce9dc69a44\"},{\"content\":{\"connectorIds\":[\"LConn1\",\"LConn2\"],\"side\":\"TOP\"},\"type\":\"ConnectorPlacement.EquallySpacedRectSide\",\"uuid\":\"3c3d5018-dce6-49a5-a481-da9d1bef79f3\"},{\"content\":{\"connectorIds\":[\"RConn1\",\"RConn2\"],\"side\":\"BOTTOM\"},\"type\":\"ConnectorPlacement.EquallySpacedRectSide\",\"uuid\":\"784ed6f0-011d-4b8b-967f-9fa51b650c0c\"}]},\"type\":\"ConnectorPlacement.EquallySpacedConnector\",\"uuid\":\"e53138d9-4137-42d6-a542-1330f1bd4428\"}],\"packageUris\":[\"http://schema.mathworks.com/mf0/Connector/R2020b\"],\"version\":\"1.0\"}"
  RLC_31 : Subsystem  mask{R=R(31), L=L(31), C=C(31)}
      settings: PortSchema="{\"entries\":[{\"content\":{\"sides\":[{\"content\":{\"connectorIds\":[]},\"type\":\"ConnectorPlacement.EquallySpacedRectSide\",\"uuid\":\"60dc27b1-37aa-45ee-bf60-4a562adeaebe\"},{\"content\":{\"connectorIds\":[],\"side\":\"RIGHT\"},\"type\":\"ConnectorPlacement.EquallySpacedRectSide\",\"uuid\":\"71f27a35-0868-434d-9527-40ce9dc69a44\"},{\"content\":{\"connectorIds\":[\"LConn1\",\"LConn2\"],\"side\":\"TOP\"},\"type\":\"ConnectorPlacement.EquallySpacedRectSide\",\"uuid\":\"3c3d5018-dce6-49a5-a481-da9d1bef79f3\"},{\"content\":{\"connectorIds\":[\"RConn1\",\"RConn2\"],\"side\":\"BOTTOM\"},\"type\":\"ConnectorPlacement.EquallySpacedRectSide\",\"uuid\":\"784ed6f0-011d-4b8b-967f-9fa51b650c0c\"}]},\"type\":\"ConnectorPlacement.EquallySpacedConnector\",\"uuid\":\"e53138d9-4137-42d6-a542-1330f1bd4428\"}],\"packageUris\":[\"http://schema.mathworks.com/mf0/Connector/R2020b\"],\"version\":\"1.0\"}"
  RLC_32 : Subsystem  mask{R=R(32), L=L(32), C=C(32)}
      settings: PortSchema="{\"entries\":[{\"content\":{\"sides\":[{\"content\":{\"connectorIds\":[]},\"type\":\"ConnectorPlacement.EquallySpacedRectSide\",\"uuid\":\"60dc27b1-37aa-45ee-bf60-4a562adeaebe\"},{\"content\":{\"connectorIds\":[],\"side\":\"RIGHT\"},\"type\":\"ConnectorPlacement.EquallySpacedRectSide\",\"uuid\":\"71f27a35-0868-434d-9527-40ce9dc69a44\"},{\"content\":{\"connectorIds\":[\"LConn1\",\"LConn2\"],\"side\":\"TOP\"},\"type\":\"ConnectorPlacement.EquallySpacedRectSide\",\"uuid\":\"3c3d5018-dce6-49a5-a481-da9d1bef79f3\"},{\"content\":{\"connectorIds\":[\"RConn1\",\"RConn2\"],\"side\":\"BOTTOM\"},\"type\":\"ConnectorPlacement.EquallySpacedRectSide\",\"uuid\":\"784ed6f0-011d-4b8b-967f-9fa51b650c0c\"}]},\"type\":\"ConnectorPlacement.EquallySpacedConnector\",\"uuid\":\"e53138d9-4137-42d6-a542-1330f1bd4428\"}],\"packageUris\":[\"http://schema.mathworks.com/mf0/Connector/R2020b\"],\"version\":\"1.0\"}"
  RLC_33 : Subsystem  mask{R=R(33), L=L(33), C=C(33)}
      settings: PortSchema="{\"entries\":[{\"content\":{\"sides\":[{\"content\":{\"connectorIds\":[]},\"type\":\"ConnectorPlacement.EquallySpacedRectSide\",\"uuid\":\"60dc27b1-37aa-45ee-bf60-4a562adeaebe\"},{\"content\":{\"connectorIds\":[],\"side\":\"RIGHT\"},\"type\":\"ConnectorPlacement.EquallySpacedRectSide\",\"uuid\":\"71f27a35-0868-434d-9527-40ce9dc69a44\"},{\"content\":{\"connectorIds\":[\"LConn1\",\"LConn2\"],\"side\":\"TOP\"},\"type\":\"ConnectorPlacement.EquallySpacedRectSide\",\"uuid\":\"3c3d5018-dce6-49a5-a481-da9d1bef79f3\"},{\"content\":{\"connectorIds\":[\"RConn1\",\"RConn2\"],\"side\":\"BOTTOM\"},\"type\":\"ConnectorPlacement.EquallySpacedRectSide\",\"uuid\":\"784ed6f0-011d-4b8b-967f-9fa51b650c0c\"}]},\"type\":\"ConnectorPlacement.EquallySpacedConnector\",\"uuid\":\"e53138d9-4137-42d6-a542-1330f1bd4428\"}],\"packageUris\":[\"http://schema.mathworks.com/mf0/Connector/R2020b\"],\"version\":\"1.0\"}"
  RLC_34 : Subsystem  mask{R=R(34), L=L(34), C=C(34)}
      settings: PortSchema="{\"entries\":[{\"content\":{\"sides\":[{\"content\":{\"connectorIds\":[]},\"type\":\"ConnectorPlacement.EquallySpacedRectSide\",\"uuid\":\"60dc27b1-37aa-45ee-bf60-4a562adeaebe\"},{\"content\":{\"connectorIds\":[],\"side\":\"RIGHT\"},\"type\":\"ConnectorPlacement.EquallySpacedRectSide\",\"uuid\":\"71f27a35-0868-434d-9527-40ce9dc69a44\"},{\"content\":{\"connectorIds\":[\"LConn1\",\"LConn2\"],\"side\":\"TOP\"},\"type\":\"ConnectorPlacement.EquallySpacedRectSide\",\"uuid\":\"3c3d5018-dce6-49a5-a481-da9d1bef79f3\"},{\"content\":{\"connectorIds\":[\"RConn1\",\"RConn2\"],\"side\":\"BOTTOM\"},\"type\":\"ConnectorPlacement.EquallySpacedRectSide\",\"uuid\":\"784ed6f0-011d-4b8b-967f-9fa51b650c0c\"}]},\"type\":\"ConnectorPlacement.EquallySpacedConnector\",\"uuid\":\"e53138d9-4137-42d6-a542-1330f1bd4428\"}],\"packageUris\":[\"http://schema.mathworks.com/mf0/Connector/R2020b\"],\"version\":\"1.0\"}"
  RLC_35 : Subsystem  mask{R=R(35), L=L(35), C=C(35)}
      settings: PortSchema="{\"entries\":[{\"content\":{\"sides\":[{\"content\":{\"connectorIds\":[]},\"type\":\"ConnectorPlacement.EquallySpacedRectSide\",\"uuid\":\"60dc27b1-37aa-45ee-bf60-4a562adeaebe\"},{\"content\":{\"connectorIds\":[],\"side\":\"RIGHT\"},\"type\":\"ConnectorPlacement.EquallySpacedRectSide\",\"uuid\":\"71f27a35-0868-434d-9527-40ce9dc69a44\"},{\"content\":{\"connectorIds\":[\"LConn1\",\"LConn2\"],\"side\":\"TOP\"},\"type\":\"ConnectorPlacement.EquallySpacedRectSide\",\"uuid\":\"3c3d5018-dce6-49a5-a481-da9d1bef79f3\"},{\"content\":{\"connectorIds\":[\"RConn1\",\"RConn2\"],\"side\":\"BOTTOM\"},\"type\":\"ConnectorPlacement.EquallySpacedRectSide\",\"uuid\":\"784ed6f0-011d-4b8b-967f-9fa51b650c0c\"}]},\"type\":\"ConnectorPlacement.EquallySpacedConnector\",\"uuid\":\"e53138d9-4137-42d6-a542-1330f1bd4428\"}],\"packageUris\":[\"http://schema.mathworks.com/mf0/Connector/R2020b\"],\"version\":\"1.0\"}"
  RLC_36 : Subsystem  mask{R=R(11), L=L(11), C=C(11)}
  RLC_37 : Subsystem  mask{R=R(12), L=L(12), C=C(12)}
  RLC_38 : Subsystem  mask{R=R(13), L=L(13), C=C(13)}
  RLC_39 : Subsystem  mask{R=R(14), L=L(14), C=C(14)}
  RLC_4 : Subsystem  mask{R=R(4), L=L(4), C=C(4)}
  RLC_40 : Subsystem  mask{R=R(15), L=L(15), C=C(15)}
  RLC_41 : Subsystem  mask{R=R(16), L=L(16), C=C(16)}
  RLC_42 : Subsystem  mask{R=R(17), L=L(17), C=C(17)}
  RLC_43 : Subsystem  mask{R=R(18), L=L(18), C=C(18)}
  RLC_44 : Subsystem  mask{R=R(19), L=L(19), C=C(19)}
  RLC_45 : Subsystem  mask{R=R(20), L=L(20), C=C(20)}
  RLC_46 : Subsystem  mask{R=R(21), L=L(21), C=C(21)}
  RLC_47 : Subsystem  mask{R=R(22), L=L(22), C=C(22)}
  RLC_48 : Subsystem  mask{R=R(23), L=L(23), C=C(23)}
  RLC_49 : Subsystem  mask{R=R(24), L=L(24), C=C(24)}
  RLC_5 : Subsystem  mask{R=R(5), L=L(5), C=C(5)}
      settings: PortSchema="{\"entries\":[{\"content\":{\"sides\":[{\"content\":{\"connectorIds\":[]},\"type\":\"ConnectorPlacement.EquallySpacedRectSide\",\"uuid\":\"60dc27b1-37aa-45ee-bf60-4a562adeaebe\"},{\"content\":{\"connectorIds\":[],\"side\":\"RIGHT\"},\"type\":\"ConnectorPlacement.EquallySpacedRectSide\",\"uuid\":\"71f27a35-0868-434d-9527-40ce9dc69a44\"},{\"content\":{\"connectorIds\":[\"LConn1\",\"LConn2\"],\"side\":\"TOP\"},\"type\":\"ConnectorPlacement.EquallySpacedRectSide\",\"uuid\":\"3c3d5018-dce6-49a5-a481-da9d1bef79f3\"},{\"content\":{\"connectorIds\":[\"RConn1\",\"RConn2\"],\"side\":\"BOTTOM\"},\"type\":\"ConnectorPlacement.EquallySpacedRectSide\",\"uuid\":\"784ed6f0-011d-4b8b-967f-9fa51b650c0c\"}]},\"type\":\"ConnectorPlacement.EquallySpacedConnector\",\"uuid\":\"e53138d9-4137-42d6-a542-1330f1bd4428\"}],\"packageUris\":[\"http://schema.mathworks.com/mf0/Connector/R2020b\"],\"version\":\"1.0\"}"
  RLC_50 : Subsystem  mask{R=R(25), L=L(25), C=C(25)}
  RLC_51 : Subsystem  mask{R=R(26), L=L(26), C=C(26)}
  RLC_52 : Subsystem  mask{R=R(27), L=L(27), C=C(27)}
      settings: PortSchema="{\"entries\":[{\"content\":{\"sides\":[{\"content\":{\"connectorIds\":[]},\"type\":\"ConnectorPlacement.EquallySpacedRectSide\",\"uuid\":\"60dc27b1-37aa-45ee-bf60-4a562adeaebe\"},{\"content\":{\"connectorIds\":[],\"side\":\"RIGHT\"},\"type\":\"ConnectorPlacement.EquallySpacedRectSide\",\"uuid\":\"71f27a35-0868-434d-9527-40ce9dc69a44\"},{\"content\":{\"connectorIds\":[\"LConn1\",\"LConn2\"],\"side\":\"TOP\"},\"type\":\"ConnectorPlacement.EquallySpacedRectSide\",\"uuid\":\"3c3d5018-dce6-49a5-a481-da9d1bef79f3\"},{\"content\":{\"connectorIds\":[\"RConn1\",\"RConn2\"],\"side\":\"BOTTOM\"},\"type\":\"ConnectorPlacement.EquallySpacedRectSide\",\"uuid\":\"784ed6f0-011d-4b8b-967f-9fa51b650c0c\"}]},\"type\":\"ConnectorPlacement.EquallySpacedConnector\",\"uuid\":\"e53138d9-4137-42d6-a542-1330f1bd4428\"}],\"packageUris\":[\"http://schema.mathworks.com/mf0/Connector/R2020b\"],\"version\":\"1.0\"}"
  RLC_53 : Subsystem  mask{R=R(28), L=L(28), C=C(28)}
      settings: PortSchema="{\"entries\":[{\"content\":{\"sides\":[{\"content\":{\"connectorIds\":[]},\"type\":\"ConnectorPlacement.EquallySpacedRectSide\",\"uuid\":\"60dc27b1-37aa-45ee-bf60-4a562adeaebe\"},{\"content\":{\"connectorIds\":[],\"side\":\"RIGHT\"},\"type\":\"ConnectorPlacement.EquallySpacedRectSide\",\"uuid\":\"71f27a35-0868-434d-9527-40ce9dc69a44\"},{\"content\":{\"connectorIds\":[\"LConn1\",\"LConn2\"],\"side\":\"TOP\"},\"type\":\"ConnectorPlacement.EquallySpacedRectSide\",\"uuid\":\"3c3d5018-dce6-49a5-a481-da9d1bef79f3\"},{\"content\":{\"connectorIds\":[\"RConn1\",\"RConn2\"],\"side\":\"BOTTOM\"},\"type\":\"ConnectorPlacement.EquallySpacedRectSide\",\"uuid\":\"784ed6f0-011d-4b8b-967f-9fa51b650c0c\"}]},\"type\":\"ConnectorPlacement.EquallySpacedConnector\",\"uuid\":\"e53138d9-4137-42d6-a542-1330f1bd4428\"}],\"packageUris\":[\"http://schema.mathworks.com/mf0/Connector/R2020b\"],\"version\":\"1.0\"}"
  RLC_54 : Subsystem  mask{R=R(29), L=L(29), C=C(29)}
      settings: PortSchema="{\"entries\":[{\"content\":{\"sides\":[{\"content\":{\"connectorIds\":[]},\"type\":\"ConnectorPlacement.EquallySpacedRectSide\",\"uuid\":\"60dc27b1-37aa-45ee-bf60-4a562adeaebe\"},{\"content\":{\"connectorIds\":[],\"side\":\"RIGHT\"},\"type\":\"ConnectorPlacement.EquallySpacedRectSide\",\"uuid\":\"71f27a35-0868-434d-9527-40ce9dc69a44\"},{\"content\":{\"connectorIds\":[\"LConn1\",\"LConn2\"],\"side\":\"TOP\"},\"type\":\"ConnectorPlacement.EquallySpacedRectSide\",\"uuid\":\"3c3d5018-dce6-49a5-a481-da9d1bef79f3\"},{\"content\":{\"connectorIds\":[\"RConn1\",\"RConn2\"],\"side\":\"BOTTOM\"},\"type\":\"ConnectorPlacement.EquallySpacedRectSide\",\"uuid\":\"784ed6f0-011d-4b8b-967f-9fa51b650c0c\"}]},\"type\":\"ConnectorPlacement.EquallySpacedConnector\",\"uuid\":\"e53138d9-4137-42d6-a542-1330f1bd4428\"}],\"packageUris\":[\"http://schema.mathworks.com/mf0/Connector/R2020b\"],\"version\":\"1.0\"}"
  RLC_55 : Subsystem  mask{R=R(30), L=L(30), C=C(30)}
      settings: PortSchema="{\"entries\":[{\"content\":{\"sides\":[{\"content\":{\"connectorIds\":[]},\"type\":\"ConnectorPlacement.EquallySpacedRectSide\",\"uuid\":\"60dc27b1-37aa-45ee-bf60-4a562adeaebe\"},{\"content\":{\"connectorIds\":[],\"side\":\"RIGHT\"},\"type\":\"ConnectorPlacement.EquallySpacedRectSide\",\"uuid\":\"71f27a35-0868-434d-9527-40ce9dc69a44\"},{\"content\":{\"connectorIds\":[\"LConn1\",\"LConn2\"],\"side\":\"TOP\"},\"type\":\"ConnectorPlacement.EquallySpacedRectSide\",\"uuid\":\"3c3d5018-dce6-49a5-a481-da9d1bef79f3\"},{\"content\":{\"connectorIds\":[\"RConn1\",\"RConn2\"],\"side\":\"BOTTOM\"},\"type\":\"ConnectorPlacement.EquallySpacedRectSide\",\"uuid\":\"784ed6f0-011d-4b8b-967f-9fa51b650c0c\"}]},\"type\":\"ConnectorPlacement.EquallySpacedConnector\",\"uuid\":\"e53138d9-4137-42d6-a542-1330f1bd4428\"}],\"packageUris\":[\"http://schema.mathworks.com/mf0/Connector/R2020b\"],\"version\":\"1.0\"}"
  RLC_56 : Subsystem  mask{R=R(31), L=L(31), C=C(31)}
      settings: PortSchema="{\"entries\":[{\"content\":{\"sides\":[{\"content\":{\"connectorIds\":[]},\"type\":\"ConnectorPlacement.EquallySpacedRectSide\",\"uuid\":\"60dc27b1-37aa-45ee-bf60-4a562adeaebe\"},{\"content\":{\"connectorIds\":[],\"side\":\"RIGHT\"},\"type\":\"ConnectorPlacement.EquallySpacedRectSide\",\"uuid\":\"71f27a35-0868-434d-9527-40ce9dc69a44\"},{\"content\":{\"connectorIds\":[\"LConn1\",\"LConn2\"],\"side\":\"TOP\"},\"type\":\"ConnectorPlacement.EquallySpacedRectSide\",\"uuid\":\"3c3d5018-dce6-49a5-a481-da9d1bef79f3\"},{\"content\":{\"connectorIds\":[\"RConn1\",\"RConn2\"],\"side\":\"BOTTOM\"},\"type\":\"ConnectorPlacement.EquallySpacedRectSide\",\"uuid\":\"784ed6f0-011d-4b8b-967f-9fa51b650c0c\"}]},\"type\":\"ConnectorPlacement.EquallySpacedConnector\",\"uuid\":\"e53138d9-4137-42d6-a542-1330f1bd4428\"}],\"packageUris\":[\"http://schema.mathworks.com/mf0/Connector/R2020b\"],\"version\":\"1.0\"}"
  RLC_57 : Subsystem  mask{R=R(32), L=L(32), C=C(32)}
      settings: PortSchema="{\"entries\":[{\"content\":{\"sides\":[{\"content\":{\"connectorIds\":[]},\"type\":\"ConnectorPlacement.EquallySpacedRectSide\",\"uuid\":\"60dc27b1-37aa-45ee-bf60-4a562adeaebe\"},{\"content\":{\"connectorIds\":[],\"side\":\"RIGHT\"},\"type\":\"ConnectorPlacement.EquallySpacedRectSide\",\"uuid\":\"71f27a35-0868-434d-9527-40ce9dc69a44\"},{\"content\":{\"connectorIds\":[\"LConn1\",\"LConn2\"],\"side\":\"TOP\"},\"type\":\"ConnectorPlacement.EquallySpacedRectSide\",\"uuid\":\"3c3d5018-dce6-49a5-a481-da9d1bef79f3\"},{\"content\":{\"connectorIds\":[\"RConn1\",\"RConn2\"],\"side\":\"BOTTOM\"},\"type\":\"ConnectorPlacement.EquallySpacedRectSide\",\"uuid\":\"784ed6f0-011d-4b8b-967f-9fa51b650c0c\"}]},\"type\":\"ConnectorPlacement.EquallySpacedConnector\",\"uuid\":\"e53138d9-4137-42d6-a542-1330f1bd4428\"}],\"packageUris\":[\"http://schema.mathworks.com/mf0/Connector/R2020b\"],\"version\":\"1.0\"}"
  RLC_58 : Subsystem  mask{R=R(33), L=L(33), C=C(33)}
      settings: PortSchema="{\"entries\":[{\"content\":{\"sides\":[{\"content\":{\"connectorIds\":[]},\"type\":\"ConnectorPlacement.EquallySpacedRectSide\",\"uuid\":\"60dc27b1-37aa-45ee-bf60-4a562adeaebe\"},{\"content\":{\"connectorIds\":[],\"side\":\"RIGHT\"},\"type\":\"ConnectorPlacement.EquallySpacedRectSide\",\"uuid\":\"71f27a35-0868-434d-9527-40ce9dc69a44\"},{\"content\":{\"connectorIds\":[\"LConn1\",\"LConn2\"],\"side\":\"TOP\"},\"type\":\"ConnectorPlacement.EquallySpacedRectSide\",\"uuid\":\"3c3d5018-dce6-49a5-a481-da9d1bef79f3\"},{\"content\":{\"connectorIds\":[\"RConn1\",\"RConn2\"],\"side\":\"BOTTOM\"},\"type\":\"ConnectorPlacement.EquallySpacedRectSide\",\"uuid\":\"784ed6f0-011d-4b8b-967f-9fa51b650c0c\"}]},\"type\":\"ConnectorPlacement.EquallySpacedConnector\",\"uuid\":\"e53138d9-4137-42d6-a542-1330f1bd4428\"}],\"packageUris\":[\"http://schema.mathworks.com/mf0/Connector/R2020b\"],\"version\":\"1.0\"}"
  RLC_59 : Subsystem  mask{R=R(34), L=L(34), C=C(34)}
      settings: PortSchema="{\"entries\":[{\"content\":{\"sides\":[{\"content\":{\"connectorIds\":[]},\"type\":\"ConnectorPlacement.EquallySpacedRectSide\",\"uuid\":\"60dc27b1-37aa-45ee-bf60-4a562adeaebe\"},{\"content\":{\"connectorIds\":[],\"side\":\"RIGHT\"},\"type\":\"ConnectorPlacement.EquallySpacedRectSide\",\"uuid\":\"71f27a35-0868-434d-9527-40ce9dc69a44\"},{\"content\":{\"connectorIds\":[\"LConn1\",\"LConn2\"],\"side\":\"TOP\"},\"type\":\"ConnectorPlacement.EquallySpacedRectSide\",\"uuid\":\"3c3d5018-dce6-49a5-a481-da9d1bef79f3\"},{\"content\":{\"connectorIds\":[\"RConn1\",\"RConn2\"],\"side\":\"BOTTOM\"},\"type\":\"ConnectorPlacement.EquallySpacedRectSide\",\"uuid\":\"784ed6f0-011d-4b8b-967f-9fa51b650c0c\"}]},\"type\":\"ConnectorPlacement.EquallySpacedConnector\",\"uuid\":\"e53138d9-4137-42d6-a542-1330f1bd4428\"}],\"packageUris\":[\"http://schema.mathworks.com/mf0/Connector/R2020b\"],\"version\":\"1.0\"}"
  RLC_6 : Subsystem  mask{R=R(6), L=L(6), C=C(6)}
      settings: PortSchema="{\"entries\":[{\"content\":{\"sides\":[{\"content\":{\"connectorIds\":[]},\"type\":\"ConnectorPlacement.EquallySpacedRectSide\",\"uuid\":\"60dc27b1-37aa-45ee-bf60-4a562adeaebe\"},{\"content\":{\"connectorIds\":[],\"side\":\"RIGHT\"},\"type\":\"ConnectorPlacement.EquallySpacedRectSide\",\"uuid\":\"71f27a35-0868-434d-9527-40ce9dc69a44\"},{\"content\":{\"connectorIds\":[\"LConn1\",\"LConn2\"],\"side\":\"TOP\"},\"type\":\"ConnectorPlacement.EquallySpacedRectSide\",\"uuid\":\"3c3d5018-dce6-49a5-a481-da9d1bef79f3\"},{\"content\":{\"connectorIds\":[\"RConn1\",\"RConn2\"],\"side\":\"BOTTOM\"},\"type\":\"ConnectorPlacement.EquallySpacedRectSide\",\"uuid\":\"784ed6f0-011d-4b8b-967f-9fa51b650c0c\"}]},\"type\":\"ConnectorPlacement.EquallySpacedConnector\",\"uuid\":\"e53138d9-4137-42d6-a542-1330f1bd4428\"}],\"packageUris\":[\"http://schema.mathworks.com/mf0/Connector/R2020b\"],\"version\":\"1.0\"}"
  RLC_60 : Subsystem  mask{R=R(60), L=L(60), C=C(60)}
  RLC_61 : Subsystem  mask{R=R(61), L=L(61), C=C(61)}
  RLC_62 : Subsystem  mask{R=R(60), L=L(60), C=C(60)}
  RLC_63 : Subsystem  mask{R=R(63), L=L(63), C=C(63)}
  RLC_64 : Subsystem  mask{R=R(64), L=L(64), C=C(64)}
  RLC_65 : Subsystem  mask{R=R(65), L=L(65), C=C(65)}
  RLC_66 : Subsystem  mask{R=R(66), L=L(66), C=C(66)}
  RLC_67 : Subsystem  mask{R=R(67), L=L(67), C=C(67)}
  RLC_68 : Subsystem  mask{R=R(68), L=L(68), C=C(68)}
  RLC_69 : Subsystem  mask{R=R(69), L=L(69), C=C(69)}
  RLC_7 : Subsystem  mask{R=R(7), L=L(7), C=C(7)}
      settings: PortSchema="{\"entries\":[{\"content\":{\"sides\":[{\"content\":{\"connectorIds\":[]},\"type\":\"ConnectorPlacement.EquallySpacedRectSide\",\"uuid\":\"60dc27b1-37aa-45ee-bf60-4a562adeaebe\"},{\"content\":{\"connectorIds\":[],\"side\":\"RIGHT\"},\"type\":\"ConnectorPlacement.EquallySpacedRectSide\",\"uuid\":\"71f27a35-0868-434d-9527-40ce9dc69a44\"},{\"content\":{\"connectorIds\":[\"LConn1\",\"LConn2\"],\"side\":\"TOP\"},\"type\":\"ConnectorPlacement.EquallySpacedRectSide\",\"uuid\":\"3c3d5018-dce6-49a5-a481-da9d1bef79f3\"},{\"content\":{\"connectorIds\":[\"RConn1\",\"RConn2\"],\"side\":\"BOTTOM\"},\"type\":\"ConnectorPlacement.EquallySpacedRectSide\",\"uuid\":\"784ed6f0-011d-4b8b-967f-9fa51b650c0c\"}]},\"type\":\"ConnectorPlacement.EquallySpacedConnector\",\"uuid\":\"e53138d9-4137-42d6-a542-1330f1bd4428\"}],\"packageUris\":[\"http://schema.mathworks.com/mf0/Connector/R2020b\"],\"version\":\"1.0\"}"
  RLC_70 : Subsystem  mask{R=R(70), L=L(70), C=C(70)}
  RLC_71 : Subsystem  mask{R=R(71), L=L(71), C=C(71)}
  RLC_72 : Subsystem  mask{R=R(72), L=L(72), C=C(72)}
  RLC_73 : Subsystem  mask{R=R(73), L=L(73), C=C(73)}
  RLC_74 : Subsystem  mask{R=R(74), L=L(74), C=C(74)}
  RLC_75 : Subsystem  mask{R=R(75), L=L(75), C=C(75)}
  RLC_76 : Subsystem  mask{R=R(76), L=L(76), C=C(76)}
  RLC_77 : Subsystem  mask{R=R(77), L=L(77), C=C(77)}
  RLC_78 : Subsystem  mask{R=R(78), L=L(78), C=C(78)}
  RLC_79 : Subsystem  mask{R=R(79), L=L(79), C=C(79)}
  RLC_8 : Subsystem  mask{R=R(8), L=L(8), C=C(8)}
      settings: PortSchema="{\"entries\":[{\"content\":{\"sides\":[{\"content\":{\"connectorIds\":[]},\"type\":\"ConnectorPlacement.EquallySpacedRectSide\",\"uuid\":\"60dc27b1-37aa-45ee-bf60-4a562adeaebe\"},{\"content\":{\"connectorIds\":[],\"side\":\"RIGHT\"},\"type\":\"ConnectorPlacement.EquallySpacedRectSide\",\"uuid\":\"71f27a35-0868-434d-9527-40ce9dc69a44\"},{\"content\":{\"connectorIds\":[\"LConn1\",\"LConn2\"],\"side\":\"TOP\"},\"type\":\"ConnectorPlacement.EquallySpacedRectSide\",\"uuid\":\"3c3d5018-dce6-49a5-a481-da9d1bef79f3\"},{\"content\":{\"connectorIds\":[\"RConn1\",\"RConn2\"],\"side\":\"BOTTOM\"},\"type\":\"ConnectorPlacement.EquallySpacedRectSide\",\"uuid\":\"784ed6f0-011d-4b8b-967f-9fa51b650c0c\"}]},\"type\":\"ConnectorPlacement.EquallySpacedConnector\",\"uuid\":\"e53138d9-4137-42d6-a542-1330f1bd4428\"}],\"packageUris\":[\"http://schema.mathworks.com/mf0/Connector/R2020b\"],\"version\":\"1.0\"}"
  RLC_80 : Subsystem  mask{R=R(80), L=L(80), C=C(80)}
  RLC_81 : Subsystem  mask{R=R(81), L=L(81), C=C(81)}
  RLC_82 : Subsystem  mask{R=R(82), L=L(82), C=C(82)}
  RLC_83 : Subsystem  mask{R=R(83), L=L(83), C=C(83)}
  RLC_84 : Subsystem  mask{R=R(84), L=L(84), C=C(84)}
  RLC_85 : Subsystem  mask{R=R(85), L=L(85), C=C(85)}
  RLC_86 : Subsystem  mask{R=R(86), L=L(86), C=C(86)}
  RLC_87 : Subsystem  mask{R=R(87), L=L(87), C=C(87)}
  RLC_88 : Subsystem  mask{R=R(88), L=L(88), C=C(88)}
  RLC_89 : Subsystem  mask{R=R(89), L=L(89), C=C(89)}
  RLC_9 : Subsystem  mask{R=R(9), L=L(9), C=C(9)}
      settings: PortSchema="{\"entries\":[{\"content\":{\"sides\":[{\"content\":{\"connectorIds\":[]},\"type\":\"ConnectorPlacement.EquallySpacedRectSide\",\"uuid\":\"60dc27b1-37aa-45ee-bf60-4a562adeaebe\"},{\"content\":{\"connectorIds\":[],\"side\":\"RIGHT\"},\"type\":\"ConnectorPlacement.EquallySpacedRectSide\",\"uuid\":\"71f27a35-0868-434d-9527-40ce9dc69a44\"},{\"content\":{\"connectorIds\":[\"LConn1\",\"LConn2\"],\"side\":\"TOP\"},\"type\":\"ConnectorPlacement.EquallySpacedRectSide\",\"uuid\":\"3c3d5018-dce6-49a5-a481-da9d1bef79f3\"},{\"content\":{\"connectorIds\":[\"RConn1\",\"RConn2\"],\"side\":\"BOTTOM\"},\"type\":\"ConnectorPlacement.EquallySpacedRectSide\",\"uuid\":\"784ed6f0-011d-4b8b-967f-9fa51b650c0c\"}]},\"type\":\"ConnectorPlacement.EquallySpacedConnector\",\"uuid\":\"e53138d9-4137-42d6-a542-1330f1bd4428\"}],\"packageUris\":[\"http://schema.mathworks.com/mf0/Connector/R2020b\"],\"version\":\"1.0\"}"
  RLC_90 : Subsystem  mask{R=R(90), L=L(90), C=C(90)}
  RLC_91 : Subsystem  mask{R=R(71), L=L(71), C=C(71)}
  RLC_92 : Subsystem  mask{R=R(72), L=L(72), C=C(72)}
  RLC_93 : Subsystem  mask{R=R(73), L=L(73), C=C(73)}
  RLC_94 : Subsystem  mask{R=R(74), L=L(74), C=C(74)}
  RLC_95 : Subsystem  mask{R=R(75), L=L(75), C=C(75)}
  RLC_96 : Subsystem  mask{R=R(76), L=L(76), C=C(76)}
  RLC_97 : Subsystem  mask{R=R(77), L=L(77), C=C(77)}
  RLC_98 : Subsystem  mask{R=R(78), L=L(78), C=C(78)}
  RLC_99 : Subsystem  mask{R=R(79), L=L(79), C=C(79)}
  R_102 : ee_lib/Passive/Resistor  R=R_82 Ohm  enable_R_tol=0  R_tol=5  tol_distribution=1  nSigma=4  enable_operating_limits=0  operating_limit_action=2  power_rating=1 W  max_working_voltage=100 V  enable_faults=ee.enum.enable.no  fault_action=simscape.enum.assert.action.none  R_faulted=inf Ohm  fault_trigger=ee.enum.faults.faultTrigger.temporal  t_fault=1 s  max_permissible_current=1 A  t_fail_on_current=1 s  noise_mode=0  Tdevice=25 degC  sample_time=1e-3 s  repeatability=1  user_seed=0  auto_seed=4100311965  faulted_specify=off  faulted_priority=None  faulted=0  power_derating_T1=70 degC  power_derating_T2=155 degC  operating_temperature_range_vec=[-50, 150] degC  alpha=3.93e-3 1/K  Tmeas=25 degC  thermal_mass=100 J/K  temperature_specify=off  temperature_priority=High  temperature=298.15 K  temperature_nominal_specify=off  temperature_nominal_unit=K  temperature_nominal_value=1
  R_105 : ee_lib/Passive/Resistor  R=R_105 Ohm  enable_R_tol=0  R_tol=5  tol_distribution=1  nSigma=4  enable_operating_limits=0  operating_limit_action=2  power_rating=1 W  max_working_voltage=100 V  enable_faults=ee.enum.enable.no  fault_action=simscape.enum.assert.action.none  R_faulted=inf Ohm  fault_trigger=ee.enum.faults.faultTrigger.temporal  t_fault=1 s  max_permissible_current=1 A  t_fail_on_current=1 s  noise_mode=0  Tdevice=25 degC  sample_time=1e-3 s  repeatability=1  user_seed=0  auto_seed=1102881302  faulted_specify=off  faulted_priority=None  faulted=0  power_derating_T1=70 degC  power_derating_T2=155 degC  operating_temperature_range_vec=[-50, 150] degC  alpha=3.93e-3 1/K  Tmeas=25 degC  thermal_mass=100 J/K  temperature_specify=off  temperature_priority=High  temperature=298.15 K  temperature_nominal_specify=off  temperature_nominal_unit=K  temperature_nominal_value=1
  R_107 : ee_lib/Passive/Resistor  R=R_84 Ohm  enable_R_tol=0  R_tol=5  tol_distribution=1  nSigma=4  enable_operating_limits=0  operating_limit_action=2  power_rating=1 W  max_working_voltage=100 V  enable_faults=ee.enum.enable.no  fault_action=simscape.enum.assert.action.none  R_faulted=inf Ohm  fault_trigger=ee.enum.faults.faultTrigger.temporal  t_fault=1 s  max_permissible_current=1 A  t_fail_on_current=1 s  noise_mode=0  Tdevice=25 degC  sample_time=1e-3 s  repeatability=1  user_seed=0  auto_seed=4245314326  faulted_specify=off  faulted_priority=None  faulted=0  power_derating_T1=70 degC  power_derating_T2=155 degC  operating_temperature_range_vec=[-50, 150] degC  alpha=3.93e-3 1/K  Tmeas=25 degC  thermal_mass=100 J/K  temperature_specify=off  temperature_priority=High  temperature=298.15 K  temperature_nominal_specify=off  temperature_nominal_unit=K  temperature_nominal_value=1
  R_111 : ee_lib/Passive/Resistor  R=R_88 Ohm  enable_R_tol=0  R_tol=5  tol_distribution=1  nSigma=4  enable_operating_limits=0  operating_limit_action=2  power_rating=1 W  max_working_voltage=100 V  enable_faults=ee.enum.enable.no  fault_action=simscape.enum.assert.action.none  R_faulted=inf Ohm  fault_trigger=ee.enum.faults.faultTrigger.temporal  t_fault=1 s  max_permissible_current=1 A  t_fail_on_current=1 s  noise_mode=0  Tdevice=25 degC  sample_time=1e-3 s  repeatability=1  user_seed=0  auto_seed=3445687205  faulted_specify=off  faulted_priority=None  faulted=0  power_derating_T1=70 degC  power_derating_T2=155 degC  operating_temperature_range_vec=[-50, 150] degC  alpha=3.93e-3 1/K  Tmeas=25 degC  thermal_mass=100 J/K  temperature_specify=off  temperature_priority=High  temperature=298.15 K  temperature_nominal_specify=off  temperature_nominal_unit=K  temperature_nominal_value=1
  R_113 : ee_lib/Passive/Resistor  R=R_90 Ohm  enable_R_tol=0  R_tol=5  tol_distribution=1  nSigma=4  enable_operating_limits=0  operating_limit_action=2  power_rating=1 W  max_working_voltage=100 V  enable_faults=ee.enum.enable.no  fault_action=simscape.enum.assert.action.none  R_faulted=inf Ohm  fault_trigger=ee.enum.faults.faultTrigger.temporal  t_fault=1 s  max_permissible_current=1 A  t_fail_on_current=1 s  noise_mode=0  Tdevice=25 degC  sample_time=1e-3 s  repeatability=1  user_seed=0  auto_seed=1822039845  faulted_specify=off  faulted_priority=None  faulted=0  power_derating_T1=70 degC  power_derating_T2=155 degC  operating_temperature_range_vec=[-50, 150] degC  alpha=3.93e-3 1/K  Tmeas=25 degC  thermal_mass=100 J/K  temperature_specify=off  temperature_priority=High  temperature=298.15 K  temperature_nominal_specify=off  temperature_nominal_unit=K  temperature_nominal_value=1
  R_26 : ee_lib/Passive/Resistor  R=R_26 Ohm  enable_R_tol=0  R_tol=5  tol_distribution=1  nSigma=4  enable_operating_limits=0  operating_limit_action=2  power_rating=1 W  max_working_voltage=100 V  enable_faults=ee.enum.enable.no  fault_action=simscape.enum.assert.action.none  R_faulted=inf Ohm  fault_trigger=ee.enum.faults.faultTrigger.temporal  t_fault=1 s  max_permissible_current=1 A  t_fail_on_current=1 s  noise_mode=0  Tdevice=25 degC  sample_time=1e-3 s  repeatability=1  user_seed=0  auto_seed=2846738949  faulted_specify=off  faulted_priority=None  faulted=0  power_derating_T1=70 degC  power_derating_T2=155 degC  operating_temperature_range_vec=[-50, 150] degC  alpha=3.93e-3 1/K  Tmeas=25 degC  thermal_mass=100 J/K  temperature_specify=off  temperature_priority=High  temperature=298.15 K  temperature_nominal_specify=off  temperature_nominal_unit=K  temperature_nominal_value=1
  R_29 : ee_lib/Passive/Resistor  R=R_29 Ohm  enable_R_tol=0  R_tol=5  tol_distribution=1  nSigma=4  enable_operating_limits=0  operating_limit_action=2  power_rating=1 W  max_working_voltage=100 V  enable_faults=ee.enum.enable.no  fault_action=simscape.enum.assert.action.none  R_faulted=inf Ohm  fault_trigger=ee.enum.faults.faultTrigger.temporal  t_fault=1 s  max_permissible_current=1 A  t_fail_on_current=1 s  noise_mode=0  Tdevice=25 degC  sample_time=1e-3 s  repeatability=1  user_seed=0  auto_seed=3134078215  faulted_specify=off  faulted_priority=None  faulted=0  power_derating_T1=70 degC  power_derating_T2=155 degC  operating_temperature_range_vec=[-50, 150] degC  alpha=3.93e-3 1/K  Tmeas=25 degC  thermal_mass=100 J/K  temperature_specify=off  temperature_priority=High  temperature=298.15 K  temperature_nominal_specify=off  temperature_nominal_unit=K  temperature_nominal_value=1
  R_34 : ee_lib/Passive/Resistor  R=R_34 Ohm  enable_R_tol=0  R_tol=5  tol_distribution=1  nSigma=4  enable_operating_limits=0  operating_limit_action=2  power_rating=1 W  max_working_voltage=100 V  enable_faults=ee.enum.enable.no  fault_action=simscape.enum.assert.action.none  R_faulted=inf Ohm  fault_trigger=ee.enum.faults.faultTrigger.temporal  t_fault=1 s  max_permissible_current=1 A  t_fail_on_current=1 s  noise_mode=0  Tdevice=25 degC  sample_time=1e-3 s  repeatability=1  user_seed=0  auto_seed=3256011594  faulted_specify=off  faulted_priority=None  faulted=0  power_derating_T1=70 degC  power_derating_T2=155 degC  operating_temperature_range_vec=[-50, 150] degC  alpha=3.93e-3 1/K  Tmeas=25 degC  thermal_mass=100 J/K  temperature_specify=off  temperature_priority=High  temperature=298.15 K  temperature_nominal_specify=off  temperature_nominal_unit=K  temperature_nominal_value=1
  R_35 : ee_lib/Passive/Resistor  R=R_35 Ohm  enable_R_tol=0  R_tol=5  tol_distribution=1  nSigma=4  enable_operating_limits=0  operating_limit_action=2  power_rating=1 W  max_working_voltage=100 V  enable_faults=ee.enum.enable.no  fault_action=simscape.enum.assert.action.none  R_faulted=inf Ohm  fault_trigger=ee.enum.faults.faultTrigger.temporal  t_fault=1 s  max_permissible_current=1 A  t_fail_on_current=1 s  noise_mode=0  Tdevice=25 degC  sample_time=1e-3 s  repeatability=1  user_seed=0  auto_seed=3890346746  faulted_specify=off  faulted_priority=None  faulted=0  power_derating_T1=70 degC  power_derating_T2=155 degC  operating_temperature_range_vec=[-50, 150] degC  alpha=3.93e-3 1/K  Tmeas=25 degC  thermal_mass=100 J/K  temperature_specify=off  temperature_priority=High  temperature=298.15 K  temperature_nominal_specify=off  temperature_nominal_unit=K  temperature_nominal_value=1
  R_51 : ee_lib/Passive/Resistor  R=R_26 Ohm  enable_R_tol=0  R_tol=5  tol_distribution=1  nSigma=4  enable_operating_limits=0  operating_limit_action=2  power_rating=1 W  max_working_voltage=100 V  enable_faults=ee.enum.enable.no  fault_action=simscape.enum.assert.action.none  R_faulted=inf Ohm  fault_trigger=ee.enum.faults.faultTrigger.temporal  t_fault=1 s  max_permissible_current=1 A  t_fail_on_current=1 s  noise_mode=0  Tdevice=25 degC  sample_time=1e-3 s  repeatability=1  user_seed=0  auto_seed=2807577747  faulted_specify=off  faulted_priority=None  faulted=0  power_derating_T1=70 degC  power_derating_T2=155 degC  operating_temperature_range_vec=[-50, 150] degC  alpha=3.93e-3 1/K  Tmeas=25 degC  thermal_mass=100 J/K  temperature_specify=off  temperature_priority=High  temperature=298.15 K  temperature_nominal_specify=off  temperature_nominal_unit=K  temperature_nominal_value=1
  R_54 : ee_lib/Passive/Resistor  R=R_29 Ohm  enable_R_tol=0  R_tol=5  tol_distribution=1  nSigma=4  enable_operating_limits=0  operating_limit_action=2  power_rating=1 W  max_working_voltage=100 V  enable_faults=ee.enum.enable.no  fault_action=simscape.enum.assert.action.none  R_faulted=inf Ohm  fault_trigger=ee.enum.faults.faultTrigger.temporal  t_fault=1 s  max_permissible_current=1 A  t_fail_on_current=1 s  noise_mode=0  Tdevice=25 degC  sample_time=1e-3 s  repeatability=1  user_seed=0  auto_seed=107953942  faulted_specify=off  faulted_priority=None  faulted=0  power_derating_T1=70 degC  power_derating_T2=155 degC  operating_temperature_range_vec=[-50, 150] degC  alpha=3.93e-3 1/K  Tmeas=25 degC  thermal_mass=100 J/K  temperature_specify=off  temperature_priority=High  temperature=298.15 K  temperature_nominal_specify=off  temperature_nominal_unit=K  temperature_nominal_value=1
  R_59 : ee_lib/Passive/Resistor  R=R_34 Ohm  enable_R_tol=0  R_tol=5  tol_distribution=1  nSigma=4  enable_operating_limits=0  operating_limit_action=2  power_rating=1 W  max_working_voltage=100 V  enable_faults=ee.enum.enable.no  fault_action=simscape.enum.assert.action.none  R_faulted=inf Ohm  fault_trigger=ee.enum.faults.faultTrigger.temporal  t_fault=1 s  max_permissible_current=1 A  t_fail_on_current=1 s  noise_mode=0  Tdevice=25 degC  sample_time=1e-3 s  repeatability=1  user_seed=0  auto_seed=1767780679  faulted_specify=off  faulted_priority=None  faulted=0  power_derating_T1=70 degC  power_derating_T2=155 degC  operating_temperature_range_vec=[-50, 150] degC  alpha=3.93e-3 1/K  Tmeas=25 degC  thermal_mass=100 J/K  temperature_specify=off  temperature_priority=High  temperature=298.15 K  temperature_nominal_specify=off  temperature_nominal_unit=K  temperature_nominal_value=1
  R_60 : ee_lib/Passive/Resistor  R=R_60 Ohm  enable_R_tol=0  R_tol=5  tol_distribution=1  nSigma=4  enable_operating_limits=0  operating_limit_action=2  power_rating=1 W  max_working_voltage=100 V  enable_faults=ee.enum.enable.no  fault_action=simscape.enum.assert.action.none  R_faulted=inf Ohm  fault_trigger=ee.enum.faults.faultTrigger.temporal  t_fault=1 s  max_permissible_current=1 A  t_fail_on_current=1 s  noise_mode=0  Tdevice=25 degC  sample_time=1e-3 s  repeatability=1  user_seed=0  auto_seed=2935248798  faulted_specify=off  faulted_priority=None  faulted=0  power_derating_T1=70 degC  power_derating_T2=155 degC  operating_temperature_range_vec=[-50, 150] degC  alpha=3.93e-3 1/K  Tmeas=25 degC  thermal_mass=100 J/K  temperature_specify=off  temperature_priority=High  temperature=298.15 K  temperature_nominal_specify=off  temperature_nominal_unit=K  temperature_nominal_value=1
  R_61 : ee_lib/Passive/Resistor  R=R_61 Ohm  enable_R_tol=0  R_tol=5  tol_distribution=1  nSigma=4  enable_operating_limits=0  operating_limit_action=2  power_rating=1 W  max_working_voltage=100 V  enable_faults=ee.enum.enable.no  fault_action=simscape.enum.assert.action.none  R_faulted=inf Ohm  fault_trigger=ee.enum.faults.faultTrigger.temporal  t_fault=1 s  max_permissible_current=1 A  t_fail_on_current=1 s  noise_mode=0  Tdevice=25 degC  sample_time=1e-3 s  repeatability=1  user_seed=0  auto_seed=3933054132  faulted_specify=off  faulted_priority=None  faulted=0  power_derating_T1=70 degC  power_derating_T2=155 degC  operating_temperature_range_vec=[-50, 150] degC  alpha=3.93e-3 1/K  Tmeas=25 degC  thermal_mass=100 J/K  temperature_specify=off  temperature_priority=High  temperature=298.15 K  temperature_nominal_specify=off  temperature_nominal_unit=K  temperature_nominal_value=1
  R_62 : ee_lib/Passive/Resistor  R=R_60 Ohm  enable_R_tol=0  R_tol=5  tol_distribution=1  nSigma=4  enable_operating_limits=0  operating_limit_action=2  power_rating=1 W  max_working_voltage=100 V  enable_faults=ee.enum.enable.no  fault_action=simscape.enum.assert.action.none  R_faulted=inf Ohm  fault_trigger=ee.enum.faults.faultTrigger.temporal  t_fault=1 s  max_permissible_current=1 A  t_fail_on_current=1 s  noise_mode=0  Tdevice=25 degC  sample_time=1e-3 s  repeatability=1  user_seed=0  auto_seed=3939316790  faulted_specify=off  faulted_priority=None  faulted=0  power_derating_T1=70 degC  power_derating_T2=155 degC  operating_temperature_range_vec=[-50, 150] degC  alpha=3.93e-3 1/K  Tmeas=25 degC  thermal_mass=100 J/K  temperature_specify=off  temperature_priority=High  temperature=298.15 K  temperature_nominal_specify=off  temperature_nominal_unit=K  temperature_nominal_value=1
  R_64 : ee_lib/Passive/Resistor  R=R_64 Ohm  enable_R_tol=0  R_tol=5  tol_distribution=1  nSigma=4  enable_operating_limits=0  operating_limit_action=2  power_rating=1 W  max_working_voltage=100 V  enable_faults=ee.enum.enable.no  fault_action=simscape.enum.assert.action.none  R_faulted=inf Ohm  fault_trigger=ee.enum.faults.faultTrigger.temporal  t_fault=1 s  max_permissible_current=1 A  t_fail_on_current=1 s  noise_mode=0  Tdevice=25 degC  sample_time=1e-3 s  repeatability=1  user_seed=0  auto_seed=1219698375  faulted_specify=off  faulted_priority=None  faulted=0  power_derating_T1=70 degC  power_derating_T2=155 degC  operating_temperature_range_vec=[-50, 150] degC  alpha=3.93e-3 1/K  Tmeas=25 degC  thermal_mass=100 J/K  temperature_specify=off  temperature_priority=High  temperature=298.15 K  temperature_nominal_specify=off  temperature_nominal_unit=K  temperature_nominal_value=1
  R_65 : ee_lib/Passive/Resistor  R=R_65 Ohm  enable_R_tol=0  R_tol=5  tol_distribution=1  nSigma=4  enable_operating_limits=0  operating_limit_action=2  power_rating=1 W  max_working_voltage=100 V  enable_faults=ee.enum.enable.no  fault_action=simscape.enum.assert.action.none  R_faulted=inf Ohm  fault_trigger=ee.enum.faults.faultTrigger.temporal  t_fault=1 s  max_permissible_current=1 A  t_fail_on_current=1 s  noise_mode=0  Tdevice=25 degC  sample_time=1e-3 s  repeatability=1  user_seed=0  auto_seed=3011944697  faulted_specify=off  faulted_priority=None  faulted=0  power_derating_T1=70 degC  power_derating_T2=155 degC  operating_temperature_range_vec=[-50, 150] degC  alpha=3.93e-3 1/K  Tmeas=25 degC  thermal_mass=100 J/K  temperature_specify=off  temperature_priority=High  temperature=298.15 K  temperature_nominal_specify=off  temperature_nominal_unit=K  temperature_nominal_value=1
  R_66 : ee_lib/Passive/Resistor  R=R_66 Ohm  enable_R_tol=0  R_tol=5  tol_distribution=1  nSigma=4  enable_operating_limits=0  operating_limit_action=2  power_rating=1 W  max_working_voltage=100 V  enable_faults=ee.enum.enable.no  fault_action=simscape.enum.assert.action.none  R_faulted=inf Ohm  fault_trigger=ee.enum.faults.faultTrigger.temporal  t_fault=1 s  max_permissible_current=1 A  t_fail_on_current=1 s  noise_mode=0  Tdevice=25 degC  sample_time=1e-3 s  repeatability=1  user_seed=0  auto_seed=3586425505  faulted_specify=off  faulted_priority=None  faulted=0  power_derating_T1=70 degC  power_derating_T2=155 degC  operating_temperature_range_vec=[-50, 150] degC  alpha=3.93e-3 1/K  Tmeas=25 degC  thermal_mass=100 J/K  temperature_specify=off  temperature_priority=High  temperature=298.15 K  temperature_nominal_specify=off  temperature_nominal_unit=K  temperature_nominal_value=1
  R_70 : ee_lib/Passive/Resistor  R=R_70 Ohm  enable_R_tol=0  R_tol=5  tol_distribution=1  nSigma=4  enable_operating_limits=0  operating_limit_action=2  power_rating=1 W  max_working_voltage=100 V  enable_faults=ee.enum.enable.no  fault_action=simscape.enum.assert.action.none  R_faulted=inf Ohm  fault_trigger=ee.enum.faults.faultTrigger.temporal  t_fault=1 s  max_permissible_current=1 A  t_fail_on_current=1 s  noise_mode=0  Tdevice=25 degC  sample_time=1e-3 s  repeatability=1  user_seed=0  auto_seed=1474410262  faulted_specify=off  faulted_priority=None  faulted=0  power_derating_T1=70 degC  power_derating_T2=155 degC  operating_temperature_range_vec=[-50, 150] degC  alpha=3.93e-3 1/K  Tmeas=25 degC  thermal_mass=100 J/K  temperature_specify=off  temperature_priority=High  temperature=298.15 K  temperature_nominal_specify=off  temperature_nominal_unit=K  temperature_nominal_value=1
  R_82 : ee_lib/Passive/Resistor  R=R_82 Ohm  enable_R_tol=0  R_tol=5  tol_distribution=1  nSigma=4  enable_operating_limits=0  operating_limit_action=2  power_rating=1 W  max_working_voltage=100 V  enable_faults=ee.enum.enable.no  fault_action=simscape.enum.assert.action.none  R_faulted=inf Ohm  fault_trigger=ee.enum.faults.faultTrigger.temporal  t_fault=1 s  max_permissible_current=1 A  t_fail_on_current=1 s  noise_mode=0  Tdevice=25 degC  sample_time=1e-3 s  repeatability=1  user_seed=0  auto_seed=3093088569  faulted_specify=off  faulted_priority=None  faulted=0  power_derating_T1=70 degC  power_derating_T2=155 degC  operating_temperature_range_vec=[-50, 150] degC  alpha=3.93e-3 1/K  Tmeas=25 degC  thermal_mass=100 J/K  temperature_specify=off  temperature_priority=High  temperature=298.15 K  temperature_nominal_specify=off  temperature_nominal_unit=K  temperature_nominal_value=1
  R_84 : ee_lib/Passive/Resistor  R=R_84 Ohm  enable_R_tol=0  R_tol=5  tol_distribution=1  nSigma=4  enable_operating_limits=0  operating_limit_action=2  power_rating=1 W  max_working_voltage=100 V  enable_faults=ee.enum.enable.no  fault_action=simscape.enum.assert.action.none  R_faulted=inf Ohm  fault_trigger=ee.enum.faults.faultTrigger.temporal  t_fault=1 s  max_permissible_current=1 A  t_fail_on_current=1 s  noise_mode=0  Tdevice=25 degC  sample_time=1e-3 s  repeatability=1  user_seed=0  auto_seed=305101953  faulted_specify=off  faulted_priority=None  faulted=0  power_derating_T1=70 degC  power_derating_T2=155 degC  operating_temperature_range_vec=[-50, 150] degC  alpha=3.93e-3 1/K  Tmeas=25 degC  thermal_mass=100 J/K  temperature_specify=off  temperature_priority=High  temperature=298.15 K  temperature_nominal_specify=off  temperature_nominal_unit=K  temperature_nominal_value=1
  R_88 : ee_lib/Passive/Resistor  R=R_88 Ohm  enable_R_tol=0  R_tol=5  tol_distribution=1  nSigma=4  enable_operating_limits=0  operating_limit_action=2  power_rating=1 W  max_working_voltage=100 V  enable_faults=ee.enum.enable.no  fault_action=simscape.enum.assert.action.none  R_faulted=inf Ohm  fault_trigger=ee.enum.faults.faultTrigger.temporal  t_fault=1 s  max_permissible_current=1 A  t_fail_on_current=1 s  noise_mode=0  Tdevice=25 degC  sample_time=1e-3 s  repeatability=1  user_seed=0  auto_seed=3791758643  faulted_specify=off  faulted_priority=None  faulted=0  power_derating_T1=70 degC  power_derating_T2=155 degC  operating_temperature_range_vec=[-50, 150] degC  alpha=3.93e-3 1/K  Tmeas=25 degC  thermal_mass=100 J/K  temperature_specify=off  temperature_priority=High  temperature=298.15 K  temperature_nominal_specify=off  temperature_nominal_unit=K  temperature_nominal_value=1
  R_90 : ee_lib/Passive/Resistor  R=R_90 Ohm  enable_R_tol=0  R_tol=5  tol_distribution=1  nSigma=4  enable_operating_limits=0  operating_limit_action=2  power_rating=1 W  max_working_voltage=100 V  enable_faults=ee.enum.enable.no  fault_action=simscape.enum.assert.action.none  R_faulted=inf Ohm  fault_trigger=ee.enum.faults.faultTrigger.temporal  t_fault=1 s  max_permissible_current=1 A  t_fail_on_current=1 s  noise_mode=0  Tdevice=25 degC  sample_time=1e-3 s  repeatability=1  user_seed=0  auto_seed=3710285765  faulted_specify=off  faulted_priority=None  faulted=0  power_derating_T1=70 degC  power_derating_T2=155 degC  operating_temperature_range_vec=[-50, 150] degC  alpha=3.93e-3 1/K  Tmeas=25 degC  thermal_mass=100 J/K  temperature_specify=off  temperature_priority=High  temperature=298.15 K  temperature_nominal_specify=off  temperature_nominal_unit=K  temperature_nominal_value=1
  R_AT : fl_lib/Electrical/Electrical Elements/Resistor  R=R_AT Ohm  i_specify=off  i_priority=None  i=0 A  i_nominal_specify=off  i_nominal_unit=A  i_nominal_value=1  v_specify=off  v_priority=None  v=0 V  v_nominal_specify=off  v_nominal_unit=V  v_nominal_value=1
  R_CA : fl_lib/Electrical/Electrical Elements/Resistor  R=R_SA Ohm  i_specify=off  i_priority=None  i=0 A  i_nominal_specify=off  i_nominal_unit=A  i_nominal_value=1  v_specify=off  v_priority=None  v=0 V  v_nominal_specify=off  v_nominal_unit=V  v_nominal_value=1
  R_SA : fl_lib/Electrical/Electrical Elements/Resistor  R=R_SA Ohm  i_specify=off  i_priority=None  i=0 A  i_nominal_specify=off  i_nominal_unit=A  i_nominal_value=1  v_specify=off  v_priority=None  v=0 V  v_nominal_specify=off  v_nominal_unit=V  v_nominal_value=1
  Repeating Sequence1 : simulink/Sources/Repeating Sequence  rep_seq_t=gen_time  rep_seq_y=gen_val
  Simulink-PS Converter1 : nesl_utility/Simulink-PS Converter  PhysicalDomain=network_engine_domain  SubClassName=ps_input  LeftPortType=input  RightPortType=output  PseudoPeriodic=off  Frequencies=[]  NoiseDistribution=none  NoiseParameters=[]  Unit=1  AffineConversion=off  FilteringAndDerivatives=provide  SimscapeFilterOrder=1  InputFilterTimeConstant=0.001  UdotUserProvided=0
  Solver Configuration1 : nesl_utility/Solver Configuration  PhysicalDomain=network_engine_domain  SubClassName=solver  LeftPortType=input  RightPortType=generic  Tones=[]  Harmonics=[]  SimulateNoise=off  Profile=off  UseLocalSampling=off  EnableSwitchedLinearOptims=on  FrequencyDomain=off  UseCCode=off  RelTol=0.001  AbsTol=1e-06  MinStep=1e-09  ToWorkspace=off  RevertToSquareIcSolve=off  NumHomotopyIterations=100  PhasorMode=off  PhasorModeNumHarmonics=1  ConsistencySolver=NEWTON_FTOL  IndexReductionMethod=DerivativeReplacement  DoDC=off  ResidualTolerance=1e-9  ConsistencyTolSource=GLOBAL  ConsistencyAbsTol=0.001  ConsistencyRelTol=0.001  ConsistencyTolFactor=0.001  UseLocalSolver=off  LocalSolverChoice=NE_BACKWARD_EULER_ADVANCER  ResolveIndetEquations=on  FunctionEvalNumThread=1  LocalSolverSampleTime=.001  DoFixedCost=off  MaxNonlinIter=3  MaxModeIter=2  ComputeImpulses=off  ImpulseIterations=2  LinearAlgebra=auto  LinearAlgebraNumThread=0  EquationFormulation=NE_TIME_EF  DelaysMemoryBudget=1024  AutomaticFiltering=on  FilteringTimeConstant=0.001  PartitionStorageMethod=AS_NEEDED  PartitionMemoryBudget=1024  PartitionMethod=FAST  MultibodyUseLocalSolver=off  MultibodyLocalSolverChoice=ODE1  MultibodyLocalSolverSampleTime=0.001
  Solver Configuration2 : nesl_utility/Solver Configuration  PhysicalDomain=network_engine_domain  SubClassName=solver  LeftPortType=input  RightPortType=generic  Tones=[]  Harmonics=[]  SimulateNoise=off  Profile=off  UseLocalSampling=off  EnableSwitchedLinearOptims=on  FrequencyDomain=off  UseCCode=off  RelTol=0.001  AbsTol=0.001  MinStep=1e-09  ToWorkspace=off  RevertToSquareIcSolve=off  NumHomotopyIterations=100  PhasorMode=off  PhasorModeNumHarmonics=1  ConsistencySolver=NEWTON_FTOL  IndexReductionMethod=DerivativeReplacement  DoDC=off  ResidualTolerance=1e-09  ConsistencyTolSource=GLOBAL  ConsistencyAbsTol=0.001  ConsistencyRelTol=0.001  ConsistencyTolFactor=0.001  UseLocalSolver=off  LocalSolverChoice=NE_BACKWARD_EULER_ADVANCER  ResolveIndetEquations=on  FunctionEvalNumThread=1  LocalSolverSampleTime=0.001  DoFixedCost=off  MaxNonlinIter=3  MaxModeIter=2  ComputeImpulses=off  ImpulseIterations=2  LinearAlgebra=auto  LinearAlgebraNumThread=0  EquationFormulation=NE_TIME_EF  DelaysMemoryBudget=1024  AutomaticFiltering=on  FilteringTimeConstant=0.001  PartitionStorageMethod=AS_NEEDED  PartitionMemoryBudget=1024  PartitionMethod=ROBUST  MultibodyUseLocalSolver=off  MultibodyLocalSolverChoice=ODE1  MultibodyLocalSolverSampleTime=0.001
  Variable Capacitor1 : ee_lib/Passive/Variable Capacitor  prm=1  Cmin=1e-9 F  r=1e-6 Ohm  v0=0 V  q0=0 C
      settings: InternalSimscapePortConfiguration="{\"Bottom\":[],\"Left\":[{\"id\":\"C\",\"label\":\"C\",\"type\":\"input\"},{\"id\":\"p\",\"label\":\"+\",\"type\":\"foundation.electrical.electrical\"}],\"Right\":[{\"id\":\"n\",\"label\":\"-\",\"type\":\"foundation.electrical.electrical\"}],\"Top\":[]}"
  Voltage Source (SL) : Subsystem
      settings: CopyFcn=set_param(gcb,'LinkStatus','none')
  Voltage Sensor1 : fl_lib/Electrical/Electrical Sensors/Voltage Sensor
  wires:
  CGS to SI converter/1 -> Voltage Source (SL)/1(S)
  Divide2/1 -> Simulink-PS Converter1/1
  Repeating Sequence1/1 -> Divide2/2
  Constant5/1 -> Divide2/1
  PS-Simulink Converter2/1 -> CGS to SI converter/1
  connections:
  Solver Configuration1/RConn1 -- ERef Src/LConn1 -- RLC_1/LConn2 -- Voltage Source (SL)/RConn2
  " P_Aortic_Root"/LConn1 -- Diode55/RConn1 -- RLC_1/LConn1
  RLC_2/LConn1 -- RLC_1/RConn1 -- " P_AAsc_in"/LConn1
  RLC_2/LConn2 -- RLC_1/RConn2
  RLC_3/LConn1 -- Diode56/RConn1 -- " P_AAsc_out"/LConn1
  RLC_3/LConn2 -- RLC_2/RConn2
  RLC_91/RConn1 -- Diode10/RConn1
  RLC_4/LConn2 -- RLC_3/RConn2 -- RLC_67/LConn2 -- RLC_71/LConn2 -- RLC_91/RConn2
  RLC_5/LConn1 -- RLC_4/RConn2
  RLC_6/LConn1 -- RLC_5/RConn1
  RLC_6/LConn2 -- RLC_5/RConn2
  RLC_7/LConn1 -- RLC_6/RConn1
  RLC_7/LConn2 -- RLC_6/RConn2
  Diode32/LConn1 -- RLC_7/RConn2
  RLC_8/LConn1 -- RLC_7/RConn1 -- RLC_63/RConn2
  F_Coel/RConn1 -- Diode51/LConn1 -- F_Hep/RConn1 -- F_Lien/LConn1
  RLC_64/RConn2 -- RLC_65/RConn2 -- RLC_63/LConn2 -- RLC_66/RConn2
  R_64/LConn1 -- RLC_64/LConn1
  R_64/RConn1 -- RLC_64/LConn2
  R_65/RConn1 -- RLC_65/LConn2
  R_65/LConn1 -- RLC_65/LConn1
  R_66/RConn1 -- RLC_66/LConn2
  R_66/LConn1 -- RLC_66/LConn1
  RLC_61/RConn2 -- RLC_62/RConn2 -- RLC_8/RConn1 -- RLC_60/LConn2 -- RLC_9/LConn1
  R_61/LConn1 -- RLC_61/LConn1
  R_61/RConn1 -- RLC_61/LConn2
  R_62/RConn1 -- RLC_62/LConn2
  R_62/LConn1 -- RLC_62/LConn1
  RLC_9/RConn1 -- RLC_10/LConn1
  RLC_9/RConn2 -- RLC_10/LConn2
  R_60/LConn1 -- RLC_60/RConn1
  R_60/RConn1 -- RLC_60/RConn2
  RLC_11/LConn2 -- RLC_36/RConn2 -- RLC_10/RConn1 -- RLC_35/LConn1
  RLC_12/LConn1 -- RLC_11/RConn1
  RLC_12/LConn2 -- RLC_11/RConn2
  " P_Iliac"/LConn1 -- RLC_12/RConn1 -- RLC_13/LConn1
  RLC_13/LConn2 -- RLC_12/RConn2
  RLC_14/LConn1 -- RLC_13/RConn1
  RLC_14/LConn2 -- RLC_13/RConn2
  RLC_15/LConn2 -- RLC_14/RConn2 -- RLC_27/LConn1
  RLC_16/LConn1 -- RLC_15/RConn1
  RLC_16/LConn2 -- RLC_15/RConn2
  RLC_17/LConn1 -- RLC_16/RConn1
  RLC_17/LConn2 -- RLC_16/RConn2
  RLC_18/LConn1 -- RLC_17/RConn1
  RLC_18/LConn2 -- RLC_17/RConn2
  RLC_19/LConn1 -- Diode45/RConn1
  RLC_19/LConn2 -- RLC_18/RConn2
  RLC_20/LConn1 -- RLC_19/RConn1
  RLC_20/LConn2 -- RLC_19/RConn2
  RLC_21/LConn1 -- RLC_20/RConn1
  RLC_21/LConn2 -- RLC_20/RConn2
  Diode35/LConn1 -- Diode34/RConn1 -- Diode36/LConn1
  RLC_22/LConn2 -- RLC_21/RConn2 -- RLC_30/LConn1
  RLC_23/LConn1 -- RLC_22/RConn1
  RLC_23/LConn2 -- RLC_22/RConn2
  RLC_24/LConn1 -- RLC_23/RConn1
  RLC_24/LConn2 -- RLC_23/RConn2
  RLC_25/LConn1 -- RLC_24/RConn1
  RLC_25/LConn2 -- RLC_24/RConn2
  RLC_26/LConn1 -- RLC_25/RConn1
  RLC_26/LConn2 -- RLC_25/RConn2
  RLC_26/RConn1 -- " P_TibPost"/RConn1 -- R_26/LConn1
  RLC_26/RConn2 -- R_26/RConn1
  RLC_28/LConn1 -- RLC_27/RConn1
  RLC_28/LConn2 -- RLC_27/RConn2
  RLC_29/LConn1 -- RLC_28/RConn1
  RLC_29/LConn2 -- RLC_28/RConn2
  R_29/RConn1 -- RLC_29/RConn1
  R_29/LConn1 -- RLC_29/RConn2
  RLC_31/LConn2 -- RLC_30/RConn2
  RLC_32/LConn2 -- RLC_31/RConn2
  RLC_32/LConn1 -- RLC_31/RConn1
  RLC_31/LConn1 -- RLC_30/RConn1
  R_34/LConn1 -- " P_TibAnt"/LConn1 -- RLC_34/RConn2
  R_34/RConn1 -- RLC_34/RConn1
  RLC_34/LConn1 -- RLC_33/RConn1
  RLC_34/LConn2 -- RLC_33/RConn2
  RLC_33/LConn2 -- RLC_32/RConn2
  RLC_33/LConn1 -- RLC_32/RConn1
  RLC_37/RConn1 -- RLC_36/LConn1
  RLC_37/RConn2 -- RLC_36/LConn2
  RLC_38/RConn1 -- RLC_37/LConn1
  RLC_38/RConn2 -- RLC_37/LConn2
  RLC_39/RConn1 -- RLC_38/LConn1
  RLC_39/RConn2 -- RLC_38/LConn2
  RLC_40/RConn1 -- Diode38/RConn1
  RLC_40/RConn2 -- RLC_52/LConn1 -- RLC_39/LConn2
  RLC_41/RConn2 -- RLC_40/LConn2
  RLC_41/RConn1 -- RLC_40/LConn1
  RLC_42/RConn1 -- RLC_41/LConn1
  RLC_42/RConn2 -- RLC_41/LConn2
  RLC_43/RConn1 -- RLC_42/LConn1
  RLC_43/RConn2 -- RLC_42/LConn2
  RLC_44/RConn1 -- RLC_43/LConn1
  RLC_44/RConn2 -- RLC_43/LConn2
  RLC_45/RConn1 -- RLC_44/LConn1
  RLC_45/RConn2 -- RLC_44/LConn2
  RLC_46/RConn1 -- RLC_45/LConn1
  RLC_46/RConn2 -- RLC_45/LConn2
  RLC_55/LConn2 -- Diode43/RConn1
  RLC_47/RConn2 -- RLC_46/LConn2 -- RLC_55/LConn1
  RLC_48/RConn1 -- RLC_47/LConn1
  RLC_48/RConn2 -- RLC_47/LConn2
  RLC_49/RConn1 -- RLC_48/LConn1
  RLC_49/RConn2 -- RLC_48/LConn2
  RLC_50/RConn1 -- RLC_49/LConn1
  RLC_50/RConn2 -- RLC_49/LConn2
  RLC_51/RConn1 -- RLC_50/LConn1
  RLC_51/RConn2 -- RLC_50/LConn2
  RLC_51/LConn2 -- R_51/RConn1
  RLC_51/LConn1 -- R_51/LConn1
  R_54/RConn1 -- RLC_54/RConn1
  RLC_53/LConn2 -- RLC_52/RConn2
  RLC_53/LConn1 -- RLC_52/RConn1
  RLC_54/LConn2 -- RLC_53/RConn2
  RLC_54/LConn1 -- RLC_53/RConn1
  R_54/LConn1 -- RLC_54/RConn2
  RLC_57/LConn2 -- RLC_56/RConn2
  RLC_56/LConn1 -- RLC_55/RConn1
  RLC_56/LConn2 -- RLC_55/RConn2
  RLC_57/LConn1 -- RLC_56/RConn1
  R_59/LConn1 -- RLC_59/RConn2
  R_59/RConn1 -- RLC_59/RConn1
  RLC_58/LConn2 -- RLC_57/RConn2
  RLC_58/LConn1 -- RLC_57/RConn1
  RLC_59/LConn2 -- RLC_58/RConn2
  RLC_59/LConn1 -- RLC_58/RConn1
  RLC_68/LConn1 -- RLC_67/RConn1
  RLC_68/LConn2 -- RLC_67/RConn2
  RLC_69/LConn1 -- RLC_68/RConn1
  RLC_69/LConn2 -- RLC_68/RConn2
  RLC_70/LConn1 -- RLC_69/RConn1
  RLC_70/LConn2 -- RLC_69/RConn2
  R_70/LConn1 -- RLC_70/RConn2
  R_70/RConn1 -- " P_Carot"/RConn1 -- RLC_70/RConn1
  RLC_75/LConn2 -- RLC_74/RConn2
  RLC_82/LConn2 -- RLC_81/RConn2
  RLC_82/LConn1 -- RLC_81/RConn1
  RLC_75/LConn1 -- " P_Axi"/LConn1 -- RLC_74/RConn1
  RLC_77/LConn1 -- RLC_76/RConn1
  RLC_74/LConn2 -- RLC_73/RConn2
  RLC_80/LConn2 -- RLC_79/RConn2 -- RLC_89/LConn2
  RLC_77/LConn2 -- RLC_76/RConn2
  RLC_81/LConn2 -- RLC_80/RConn2
  F_Uln/RConn1 -- F_Uln1/LConn1 -- Diode19/LConn1
  RLC_73/LConn2 -- RLC_72/RConn2
  RLC_81/LConn1 -- RLC_80/RConn1
  RLC_78/LConn1 -- RLC_77/RConn1
  RLC_72/LConn2 -- RLC_71/RConn2 -- RLC_83/LConn2
  RLC_79/LConn2 -- RLC_78/RConn2 -- RLC_85/LConn2
  RLC_73/LConn1 -- " P_SubC"/LConn1 -- RLC_72/RConn1
  RLC_78/LConn2 -- RLC_77/RConn2
  Diode14/LConn1 -- F_SubC1/RConn1
  Diode16/LConn1 -- F_Brach/RConn1 -- F_Brach1/LConn1
  RLC_76/LConn2 -- RLC_75/RConn2
  RLC_74/LConn1 -- RLC_73/RConn1
  RLC_76/LConn1 -- RLC_75/RConn1
  RLC_82/RConn2 -- R_82/RConn1
  RLC_82/RConn1 -- R_82/LConn1 -- " P_Uln"/LConn1
  R_88/LConn1 -- RLC_88/RConn2
  R_88/RConn1 -- " P_Rad"/RConn1 -- RLC_88/RConn1
  RLC_86/LConn1 -- RLC_85/RConn1
  RLC_88/LConn2 -- RLC_87/RConn2
  RLC_87/LConn1 -- RLC_86/RConn1
  RLC_86/LConn2 -- RLC_85/RConn2
  RLC_87/LConn2 -- RLC_86/RConn2
  RLC_88/LConn1 -- RLC_87/RConn1
  RLC_84/LConn2 -- RLC_83/RConn2
  RLC_84/LConn1 -- RLC_83/RConn1
  R_84/RConn1 -- RLC_84/RConn1 -- " P_Vert"/RConn1
  R_84/LConn1 -- RLC_84/RConn2
  RLC_90/LConn1 -- RLC_89/RConn1
  RLC_90/LConn2 -- RLC_89/RConn2
  R_90/RConn1 -- " P_Vola"/RConn1 -- RLC_90/RConn1
  R_90/LConn1 -- RLC_90/RConn2
  RLC_102/RConn2 -- RLC_101/LConn2
  RLC_102/RConn1 -- RLC_101/LConn1
  RLC_95/RConn2 -- RLC_94/LConn2
  RLC_95/RConn1 -- RLC_94/LConn1
  RLC_112/LConn1 -- Diode30/RConn1
  Diode24/LConn1 -- F_Anon/RConn1 -- Diode22/LConn1
  RLC_92/RConn2 -- RLC_106/LConn2 -- RLC_103/LConn2 -- RLC_91/LConn2
  RLC_98/RConn1 -- RLC_97/LConn1
  RLC_99/RConn2 -- RLC_108/LConn2 -- RLC_98/LConn2
  RLC_94/RConn1 -- RLC_93/LConn1
  R_102/LConn1 -- RLC_102/LConn1
  RLC_93/RConn2 -- RLC_92/LConn2
  RLC_100/RConn2 -- RLC_112/LConn2 -- RLC_99/LConn2
  RLC_96/RConn1 -- RLC_95/LConn1
  RLC_93/RConn1 -- RLC_92/LConn1
  RLC_97/RConn1 -- RLC_96/LConn1
  RLC_96/RConn2 -- RLC_95/LConn2
  RLC_101/RConn2 -- RLC_100/LConn2
  RLC_94/RConn2 -- RLC_93/LConn2
  R_102/RConn1 -- RLC_102/LConn2
  RLC_101/RConn1 -- RLC_100/LConn1
  RLC_97/RConn2 -- RLC_96/LConn2
  RLC_108/LConn1 -- Diode27/RConn1
  RLC_98/RConn2 -- RLC_97/LConn2
  RLC_104/LConn1 -- RLC_103/RConn1
  RLC_104/LConn2 -- RLC_103/RConn2
  RLC_105/LConn1 -- RLC_104/RConn1
  RLC_105/LConn2 -- RLC_104/RConn2
  R_105/RConn1 -- RLC_105/RConn1
  R_105/LConn1 -- RLC_105/RConn2
  R_107/LConn1 -- RLC_107/RConn2
  RLC_107/LConn2 -- RLC_106/RConn2
  R_107/RConn1 -- RLC_107/RConn1
  RLC_107/LConn1 -- RLC_106/RConn1
  RLC_113/LConn1 -- RLC_112/RConn1
  RLC_111/LConn1 -- RLC_110/RConn1
  RLC_110/LConn1 -- RLC_109/RConn1
  R_113/LConn1 -- RLC_113/RConn2
  RLC_110/LConn2 -- RLC_109/RConn2
  R_113/RConn1 -- RLC_113/RConn1
  RLC_111/LConn2 -- RLC_110/RConn2
  R_111/RConn1 -- RLC_111/RConn1
  RLC_109/LConn1 -- RLC_108/RConn1
  RLC_113/LConn2 -- RLC_112/RConn2
  R_111/LConn1 -- RLC_111/RConn2
  RLC_109/LConn2 -- RLC_108/RConn2
  R_35/LConn1 -- RLC_35/RConn2
  R_35/RConn1 -- RLC_35/RConn1
  RLC_4/LConn1 -- Diode47/RConn1
  RLC_5/LConn2 -- " P_DescA"/LConn1 -- RLC_4/RConn1
  RLC_63/RConn1 -- Diode3/RConn1
  RLC_60/LConn1 -- Diode5/RConn1
  RLC_35/LConn2 -- Diode6/RConn1
  RLC_36/RConn1 -- F_LegR/RConn1
  Diode8/LConn1 -- F_MesI/LConn1 -- F_AbA1/RConn1 -- Diode7/LConn1
  Diode4/LConn1 -- RLC_8/RConn2
  RLC_71/LConn1 -- Diode12/RConn1
  Diode10/LConn1 -- Diode2/RConn1 -- Diode1/LConn1
  Diode11/RConn1 -- RLC_67/LConn1
  Diode11/LConn1 -- F_Arcus3/RConn1 -- F_Arcus4/LConn1
  RLC_83/LConn1 -- Diode13/RConn1
  RLC_72/LConn1 -- Diode14/RConn1
  Diode15/LConn1 -- RLC_71/RConn1
  RLC_79/LConn1 -- Diode17/RConn1
  RLC_85/LConn1 -- Diode16/RConn1
  Diode18/LConn1 -- " P_Brach"/RConn1 -- RLC_78/RConn1
  Diode21/LConn1 -- RLC_79/RConn1
  RLC_80/LConn1 -- Diode20/RConn1
  RLC_89/LConn1 -- Diode19/RConn1
  Diode23/LConn1 -- RLC_91/LConn1
  RLC_106/LConn1 -- RLC_103/LConn1 -- Diode24/RConn1
  Diode27/LConn1 -- Diode25/LConn1 -- Diode26/RConn1
  Diode26/LConn1 -- RLC_98/LConn1
  RLC_99/RConn1 -- Diode25/RConn1
  RLC_100/RConn1 -- Diode28/RConn1
  Diode28/LConn1 -- Diode30/LConn1 -- Diode29/RConn1
  Diode29/LConn1 -- RLC_99/LConn1
  RLC_27/LConn2 -- Diode31/RConn1
  " P_Po"/RConn1 -- F_Po/LConn1 -- RLC_21/RConn1
  RLC_30/LConn2 -- Diode36/RConn1
  RLC_52/LConn2 -- Diode40/RConn1
  Diode39/LConn1 -- RLC_39/LConn1
  Diode40/LConn1 -- Diode39/RConn1 -- Diode38/LConn1
  Diode42/RConn1 -- Diode41/LConn1 -- Diode43/LConn1
  Diode42/LConn1 -- RLC_46/LConn1
  RLC_47/RConn1 -- Diode41/RConn1
  F_AbA/RConn1 -- F_Rend/LConn1 -- F_MesS/LConn1 -- F_Rena/LConn1 -- Diode53/LConn1
  " P_ThA"/LConn1 -- F_ThA/RConn1 -- F_ThA1/LConn1 -- Diode3/LConn1
  Diode44/RConn1 -- RLC_8/LConn2
  Diode37/LConn1 -- Diode31/LConn1 -- Diode33/RConn1
  Diode45/LConn1 -- " P_FA"/RConn1 -- RLC_18/RConn1
  RLC_3/RConn1 -- Diode46/LConn1
  Diode46/RConn1 -- " P_AA"/LConn1 -- F_Arcus/LConn1
  F_Arcus/RConn1 -- Diode2/LConn1 -- F_Arcus2/LConn1
  F_Arcus2/RConn1 -- Diode47/LConn1
  F_Arcus3/LConn1 -- Diode1/RConn1
  F_Arcus4/RConn1 -- Diode12/LConn1
  F_SubC/LConn1 -- Diode15/RConn1
  F_SubC1/LConn1 -- F_SubC/RConn1 -- Diode13/LConn1
  Diode18/RConn1 -- F_Brach/LConn1
  F_Brach1/RConn1 -- Diode17/LConn1
  Diode21/RConn1 -- F_Uln/LConn1
  Diode20/LConn1 -- F_Uln1/RConn1
  F_ThA/LConn1 -- Diode32/RConn1
  F_ThA1/RConn1 -- Diode44/LConn1
  Diode48/RConn1 -- RLC_65/RConn1
  Diode49/LConn1 -- RLC_63/LConn1
  Diode50/RConn1 -- RLC_64/RConn1
  Diode51/RConn1 -- RLC_66/RConn1
  F_Coel/LConn1 -- Diode49/RConn1
  F_Lien/RConn1 -- Diode48/LConn1
  F_Hep/LConn1 -- Diode50/LConn1
  F_AbA/LConn1 -- Diode4/RConn1
  Diode5/LConn1 -- F_Rena/RConn1
  RLC_61/RConn1 -- Diode9/RConn1
  F_MesS/RConn1 -- Diode9/LConn1
  F_Rend/RConn1 -- Diode52/LConn1
  Diode52/RConn1 -- RLC_62/RConn1
  RLC_9/LConn2 -- Diode53/RConn1
  Diode54/LConn1 -- " P_AbA"/LConn1 -- RLC_10/RConn2
  Diode54/RConn1 -- F_AbA1/LConn1
  F_MesI/RConn1 -- Diode6/LConn1
  Diode8/RConn1 -- F_LegL/LConn1
  F_LegL/RConn1 -- RLC_11/LConn1
  F_Fem/RConn1 -- Diode33/LConn1
  RLC_14/RConn1 -- F_Fem/LConn1
  Diode37/RConn1 -- F_Fem1/LConn1
  F_Fem1/RConn1 -- RLC_15/LConn1
  F_Po/RConn1 -- Diode34/LConn1
  Diode35/RConn1 -- F_Po1/LConn1
  F_Po1/RConn1 -- RLC_22/LConn1
  F_LegR/LConn1 -- Diode7/RConn1
  Diode22/RConn1 -- F_Anon1/LConn1
  F_Anon1/RConn1 -- RLC_92/RConn1
  F_Anon/LConn1 -- Diode23/RConn1
  Electrical Reference5/LConn1 -- Voltage Sensor1/RConn2
  PS-Simulink Converter2/LConn1 -- Voltage Sensor1/RConn1
  Solver Configuration2/RConn1 -- C_CA/RConn1 -- Electrical Reference1/LConn1
  MV/RConn1 -- Voltage Sensor1/LConn1 -- F_LV/LConn1 -- Variable Capacitor1/RConn1
  C_CA/LConn1 -- R_CA/LConn1 -- R_SA/RConn1
  Simulink-PS Converter1/RConn1 -- Variable Capacitor1/LConn1
  AV/RConn1 -- R_SA/LConn1
  Electrical Reference4/LConn1 -- Variable Capacitor1/LConn2
  F_AT/RConn1 -- R_AT/LConn1
  P_SV/RConn1 -- Electrical Reference8/LConn1
  AV/LConn1 -- F_LV/RConn1
  R_AT/RConn1 -- MV/LConn1
  P_SV/LConn1 -- R_CA/RConn1
  Electrical Reference2/LConn1 -- P_AT/RConn1
  P_AT/LConn1 -- F_AT/LConn1
  RLC_2/RConn1 -- Diode56/LConn1
  Voltage Source (SL)/RConn1 -- " P_LV"/LConn1 -- Diode55/LConn1
